simulink library "xbsIndex_r4"  (Simulink 7.1)
(part 3 of 9)

  "DDS v5_0 " : S-Function  LoadFcn=xlBlockLoadCallback(gcbh);  FunctionName=sysgen  Parameters=ptable_  EnableBusSupport=off  mask(Xilinx Direct Digital Synthesizer v5_0 Block){mode_sgadvanced=, mode=Sine, neg_sin_sgadvanced=, neg_sin=off, neg_cos_sgadvanced=, neg_cos=off, channels_sgadvanced=, channels=1, output_frequency_type_sgadvanced=, output_frequency_type=Fixed, output_frequency_array=[0.0], phase_offset_type_sgadvanced=, phase_offset_type=None, phase_offset_array=[0.0], channel_port_sgadvanced=, channel_port=off, rst_sgadvanced=, rst=off, en_sgadvanced=, en=on, explicit_period_sgadvanced=, explicit_period=on, period=1, dds_clock_rate=100.0, sfdr=36.0, frequency_resolution=0.4, acc_latency_sgadvanced=, acc_latency=One Cycle, noise_shaping_sgadvanced=, noise_shaping=None, dbl_ovrd_sgadvanced=, dbl_ovrd=off, mem_type_sgadvanced=, mem_type=Distributed Memory, pipeline_sgadvanced=, pipeline=off, use_rpm_sgadvanced=, use_rpm=on, xl_use_area_sgadvanced=, xl_use_area=off, xl_area=[0,0,0,0,0,0,0], has_advanced_control=0, sggui_pos=-1,-1,-1,-1, block_type=dds, block_version=, sg_icon_stat=60,60,-1,-1,white,blue,0,07734,right,,[ ],[ ], sg_mask_display=|, sg_list_contents=, sg_blockgui_xml=}
      mask sg_mask_display=|
      | fprintf('','COMMENT: begin icon graphics');
      | patch([0 60 60 0 0 ],[0 0 60 60 0 ],[0.77 0.82 0.91 ]);
      | plot([0 60 60 0 0 ],[0 0 60 60 0 ]);
      | patch([12.2 23.76 31.76 39.76 47.76 31.76 20.2 12.2 ],[38.88 38.88 46.88 38.88 46.88 46.88 46.88 38.88 ],[1 1 1 ]);
      | patch([20.2 31.76 23.76 12.2 20.2 ],[30.88 30.88 38.88 38.88 30.88 ],[0.931 0.946 0.973 ]);
      | patch([12.2 23.76 31.76 20.2 12.2 ],[22.88 22.88 30.88 30.88 22.88 ],[1 1 1 ]);
      | patch([20.2 47.76 39.76 31.76 23.76 12.2 20.2 ],[14.88 14.88 22.88 14.88 22.88 22.88 14.88 ],[0.931 0.946 0.973 ]);
      | fprintf('','COMMENT: end icon graphics');
      | fprintf('','COMMENT: begin icon text');
      | fprintf('','COMMENT: end icon text');
      mask prompts: mode_sgadvanced ""; mode "Function"; neg_sin_sgadvanced ""; neg_sin "Negative sine"; neg_cos_sgadvanced ""; neg_cos "Negative cosine"; channels_sgadvanced ""; output_frequency_type_sgadvanced ""; output_frequency_type "Type"; output_frequency_array "Output frequency array (MHz)"; phase_offset_type_sgadvanced ""; phase_offset_type "Type"; phase_offset_array "Phase offset angle array (x 2pi Radians)"; channel_port_sgadvanced ""; channel_port "Provide channel port"; rst_sgadvanced ""; rst "Provide synchronous reset port"; en_sgadvanced ""; en "Provide enable port"; explicit_period_sgadvanced ""; explicit_period "Sample period source"; period "Explicit period"; dds_clock_rate "DDS clock rate (MHz)"; sfdr "Spurious free dynamic range (dB)"; frequency_resolution "Frequency resolution (Hz)"; acc_latency_sgadvanced ""; acc_latency "Accumulator latency"; noise_shaping_sgadvanced ""; noise_shaping "Noise Shaping"; dbl_ovrd_sgadvanced ""; dbl_ovrd "Override with doubles"; mem_type_sgadvanced ""; mem_type "Memory type"; pipeline_sgadvanced ""; pipeline "Pipeline for maximum performance"; use_rpm_sgadvanced ""; use_rpm "Use core placement information"; xl_use_area_sgadvanced ""; xl_use_area "Define FPGA area for resource estimation"; xl_area "FPGA area [slices, FFs, BRAMs, LUTs, IOBs, emb. mults, TBUFs]"; has_advanced_control ""; sggui_pos ""; block_type ""; block_version ""; sg_icon_stat ""; sg_mask_display ""; sg_list_contents ""; sg_blockgui_xml ""
      mask help: Xilinx Direct Digital Synthesizer v5_0
      mask init:
      | try
      |   tmp_gcb = gcb;
      |   tmp_gcbh = gcbh;
      |   if (strcmp('SysGenIndex',get_param(bdroot(tmp_gcbh),'tag')) && ~isempty(regexp(bdroot(tmp_gcb), '^xbs', 'once')))
      |     return;
      |   end;
      |   xlMungeMaskParams;
      |   block_config = 'sysgen_blockset:Removed_config';
      | 
      |   block_type='dds';
      | nport = get_param(gcbh, 'ports');
      | nin = nport(1);
      | nout = nport(2);
      | 
      |   serialized_declarations = '{''acc_latency''=>''Int'',''channel_port''=>''Int'',''channels''=>''Int'',''dds_clock_rate''=>''Double'',''en''=>''Int'',''explicit_period''=>''Int'',''frequency_resolution''=>''Double'',''mem_type''=>''Int'',''mode''=>''Int'',''neg_cos''=>''Int'',''neg_sin''=>''Int'',''noise_shaping''=>''Int'',''output_frequency_array''=>''DoubleVector'',''output_frequency_type''=>''Int'',''period''=>''Double'',''phase_offset_array''=>''DoubleVector'',''phase_offset_type''=>''Int'',''pipeline''=>''Int'',''rst''=>''Int'',''sfdr''=>''Double'',''use_rpm''=>''Int'',''block_type''=>''String'',''nin''=>''Double'',''nout''=>''Double''}';
      |   ptable_ = xlblockprep(get_param(tmp_gcb, 'MaskWSVariables'));
      |   try
      |     xlBlockMoveCallback(tmp_gcbh);
      |   catch 
      |      clear global xl_updateicon_recursion_guard;
      |   end;
      | catch
      |   global dbgsysgen;
      |   if(~isempty(dbgsysgen) && dbgsysgen)
      |     e = regexprep(lasterr, '\n', '\nError: ');
      |     disp(['Error: While running MaskInit code on block ' tmp_gcb ': ' e]);
      |     error(e);
      |   end
      | end
      settings: CopyFcn=xlBlockMoveCallback(gcbh);  DeleteFcn=xlDestroyGui(gcbh);  ModelCloseFcn=xlDestroyGui(gcbh);  PreSaveFcn=xlBlockPreSaveCallback(gcbh);  PostSaveFcn=xlBlockPostSaveCallback(gcbh);  DestroyFcn=xlDestroyGui(gcbh);  OpenFcn=xlOpenGui(gcbh, 'dds_gui.xml', @xlremovedenablement, -1)  CloseFcn=xlDestroyGui(gcbh);  MoveFcn=xlBlockMoveCallback(gcbh);
      mask Help: eval('');xlDoc('-book','sysgen','-topic','DDS_v5_0');
      mask StyleString: edit,popup(Sine|Cosine|Sine and Cosine),edit,checkbox,edit,checkbox,edit,popup(1|2|3|4|5|6|7|8|9|10|11|12|13|14|15|16),edit,popup(Fixed|Programmable),edit,edit,popup(Fixed|Programmable|None),edit,edit,checkbox,edit,checkbox,edit,checkbox,edit,popup(on|off),edit,edit,edit,edit,edit,popup(Zero Cycle|One Cycle),edit,popup(None|Phase dithering|Taylor series corrected|Auto),edit,checkbox,edit,popup(Distributed Memory|Block RAM),edit,checkbox,edit,checkbox,edit,checkbox,edit,edit,edit,edit,edit,edit,edit,edit,edit
      mask Display:
      | fprintf('','COMMENT: begin icon graphics');
      | patch([0 60 60 0 0 ],[0 0 60 60 0 ],[0.77 0.82 0.91 ]);
      | plot([0 60 60 0 0 ],[0 0 60 60 0 ]);
      | patch([12.2 23.76 31.76 39.76 47.76 31.76 20.2 12.2 ],[38.88 38.88 46.88 38.88 46.88 46.88 46.88 38.88 ],[1 1 1 ]);
      | patch([20.2 31.76 23.76 12.2 20.2 ],[30.88 30.88 38.88 38.88 30.88 ],[0.931 0.946 0.973 ]);
      | patch([12.2 23.76 31.76 20.2 12.2 ],[22.88 22.88 30.88 30.88 22.88 ],[1 1 1 ]);
      | patch([20.2 47.76 39.76 31.76 23.76 12.2 20.2 ],[14.88 14.88 22.88 14.88 22.88 22.88 14.88 ],[0.931 0.946 0.973 ]);
      | fprintf('','COMMENT: end icon graphics');
      | fprintf('','COMMENT: begin icon text');
      | fprintf('','COMMENT: end icon text');
  DSP48 : S-Function  LoadFcn=xlBlockLoadCallback(gcbh);  FunctionName=sysgen  Parameters=ptable_  EnableBusSupport=off  mask(Xilinx DSP48 Block){use_b_sgadvanced=, use_b=Direct from B Port, use_op_sgadvanced=, use_op=off, use_creg_sgadvanced=, use_creg=off, use_pcin_sgadvanced=, use_pcin=off, use_pcout_sgadvanced=, use_pcout=off, use_bcout_sgadvanced=, use_bcout=off, rst_all_sgadvanced=, rst_all=off, en_all_sgadvanced=, en_all=off, pipeline_a_sgadvanced=, pipeline_a=1, pipeline_b_sgadvanced=, pipeline_b=1, pipeline_c_sgadvanced=, pipeline_c=on, pipeline_p_sgadvanced=, pipeline_p=on, pipeline_mult_sgadvanced=, pipeline_mult=on, pipeline_opmode_sgadvanced=, pipeline_opmode=on, pipeline_sub_sgadvanced=, pipeline_sub=on, pipeline_carryin_sgadvanced=, pipeline_carryin=on, pipeline_carryinsel_sgadvanced=, pipeline_carryinsel=on, rst_a_sgadvanced=, rst_a=off, rst_b_sgadvanced=, rst_b=off, rst_c_sgadvanced=, rst_c=off, rst_mult_sgadvanced=, rst_mult=off, rst_p_sgadvanced=, rst_p=off, rst_carry_in_sgadvanced=, rst_carry_in=off, rst_ctrl_sgadvanced=, rst_ctrl=off, en_a_sgadvanced=, en_a=off, en_b_sgadvanced=, en_b=off, en_c_sgadvanced=, en_c=off, en_mult_sgadvanced=, en_mult=off, en_p_sgadvanced=, en_p=off, en_carry_in_sgadvanced=, en_carry_in=off, en_ctrl_sgadvanced=, en_ctrl=off, dbl_ovrd_sgadvanced=, dbl_ovrd=off, use_synth_model_sgadvanced=, use_synth_model=off, xl_useadderonly_sgadvanced=, xl_useadderonly=off, xl_use_area_sgadvanced=, xl_use_area=off, xl_area=[0,0,0,0,0,0,0], has_advanced_control=0, sggui_pos=-1,-1,-1,-1, block_type=dsp48, block_version=, sg_icon_stat=75,136,6,1,white,blue,0,aaab5c39,right,,[ ],[ ], sg_mask_display=|, sg_list_contents=, sg_blockgui_xml=}
      mask sg_mask_display=|
      | fprintf('','COMMENT: begin icon graphics');
      | patch([0 75 75 0 0 ],[0 0 136 136 0 ],[0.77 0.82 0.91 ]);
      | plot([0 75 75 0 0 ],[0 0 136 136 0 ]);
      | patch([14.75 29.2 39.2 49.2 59.2 39.2 24.75 14.75 ],[79.1 79.1 89.1 79.1 89.1 89.1 89.1 79.1 ],[1 1 1 ]);
      | patch([24.75 39.2 29.2 14.75 24.75 ],[69.1 69.1 79.1 79.1 69.1 ],[0.931 0.946 0.973 ]);
      | patch([14.75 29.2 39.2 24.75 14.75 ],[59.1 59.1 69.1 69.1 59.1 ],[1 1 1 ]);
      | patch([24.75 59.2 49.2 39.2 29.2 14.75 24.75 ],[49.1 49.1 59.1 49.1 59.1 59.1 49.1 ],[0.931 0.946 0.973 ]);
      | fprintf('','COMMENT: end icon graphics');
      | fprintf('','COMMENT: begin icon text');
      | color('black');port_label('input',1,'a');
      | color('black');port_label('input',2,'b');
      | color('black');port_label('input',3,'opmode');
      | color('black');port_label('input',4,'subtract');
      | color('black');port_label('input',5,'carry_in');
      | color('black');port_label('input',6,'carry_in_sel');
      | color('black');port_label('output',1,'p');
      | fprintf('','COMMENT: end icon text');
      mask prompts: use_b_sgadvanced ""; use_b "<tt>B</tt> or <tt>BCIN</tt> input"; use_op_sgadvanced ""; use_op "Consolidate control port (<tt>opmode</tt>, <tt>subtract</tt>, <tt>carry_in</tt>, <tt>carry_in_sel</tt>)"; use_creg_sgadvanced ""; use_creg "Provide <tt>C</tt> port"; use_pcin_sgadvanced ""; use_pcin "Provide <tt>PCIN</tt> port"; use_pcout_sgadvanced ""; use_pcout "Provide <tt>PCOUT</tt> port"; use_bcout_sgadvanced ""; use_bcout "Provide <tt>BCOUT</tt> port"; rst_all_sgadvanced ""; rst_all "Provide global reset port"; en_all_sgadvanced ""; en_all "Provide global enable port"; pipeline_a_sgadvanced ""; pipeline_a "Length of <tt>A</tt> pipeline"; pipeline_b_sgadvanced ""; pipeline_b "Length of <tt>B</tt>/<tt>BCIN</tt> pipeline"; pipeline_c_sgadvanced ""; pipeline_c "Pipeline <tt>C</tt>"; pipeline_p_sgadvanced ""; pipeline_p "Pipeline <tt>P</tt>"; pipeline_mult_sgadvanced ""; pipeline_mult "Pipeline multiplier"; pipeline_opmode_sgadvanced ""; pipeline_opmode "Pipeline <tt>opmode</tt>"; pipeline_sub_sgadvanced ""; pipeline_sub "Pipeline <tt>subtract</tt>"; pipeline_carryin_sgadvanced ""; pipeline_carryin "Pipeline carry in"; pipeline_carryinsel_sgadvanced ""; pipeline_carryinsel "Pipeline carry in sel"; rst_a_sgadvanced ""; rst_a "Reset port for <tt>A</tt>"; rst_b_sgadvanced ""; rst_b "Reset port for <tt>B</tt>/<tt>BCIN</tt>"; rst_c_sgadvanced ""; rst_c "Reset port for <tt>C</tt>"; rst_mult_sgadvanced ""; rst_mult "Reset port for multiplier"; rst_p_sgadvanced ""; rst_p "Reset port for <tt>P</tt>"; rst_carry_in_sgadvanced ""; rst_carry_in "Reset port for carry in"; rst_ctrl_sgadvanced ""; rst_ctrl "Reset port for controls<br> (<tt>opmode</tt>, <tt>subtract</tt>,<br> <tt>carry_in</tt>, <tt>carry_in_sel</tt>)"; en_a_sgadvanced ""; en_a "Enable port for <tt>A</tt>"; en_b_sgadvanced ""; en_b "Enable port for <tt>B</tt>/<tt>BCIN</tt>"; en_c_sgadvanced ""; en_c "Enable port for <tt>C</tt>"; en_mult_sgadvanced ""; en_mult "Enable port for multiplier"; en_p_sgadvanced ""; en_p "Enable port for <tt>P</tt>"; en_carry_in_sgadvanced ""; en_carry_in "Enable port for carry in"; en_ctrl_sgadvanced ""; en_ctrl "Enable port for controls<br> (<tt>opmode</tt>, <tt>subtract</tt>,<br> <tt>carry_in</tt>, <tt>carry_in_sel</tt>)"; dbl_ovrd_sgadvanced ""; dbl_ovrd "Override with doubles"; use_synth_model_sgadvanced ""; use_synth_model "Use synthesizable model"; xl_useadderonly_sgadvanced ""; xl_useadderonly "Use adder only"; xl_use_area_sgadvanced ""; xl_use_area "Define FPGA area for resource estimation"; xl_area "FPGA area [slices, FFs, BRAMs, LUTs, IOBs, emb. mults, TBUFs]"; has_advanced_control ""; sggui_pos ""; block_type ""; block_version ""; sg_icon_stat ""; sg_mask_display ""; sg_list_contents ""; sg_blockgui_xml ""
      mask help: Xilinx DSP48
      mask init:
      | try
      |   tmp_gcb = gcb;
      |   tmp_gcbh = gcbh;
      |   if (strcmp('SysGenIndex',get_param(bdroot(tmp_gcbh),'tag')) && ~isempty(regexp(bdroot(tmp_gcb), '^xbs', 'once')))
      |     return;
      |   end;
      |   xlMungeMaskParams;
      |   block_config = 'sysgen_blockset:DSP48_config';
      | 
      |   block_type='dsp48';
      | 
      |   serialized_declarations = '{''en_a''=>''Int'',''en_all''=>''Int'',''en_b''=>''Int'',''en_c''=>''Int'',''en_carry_in''=>''Int'',''en_ctrl''=>''Int'',''en_mult''=>''Int'',''en_p''=>''Int'',''pipeline_a''=>''Int'',''pipeline_b''=>''Int'',''pipeline_c''=>''Int'',''pipeline_carryin''=>''Int'',''pipeline_carryinsel''=>''Int'',''pipeline_mult''=>''Int'',''pipeline_opmode''=>''Int'',''pipeline_p''=>''Int'',''pipeline_sub''=>''Int'',''rst_a''=>''Int'',''rst_all''=>''Int'',''rst_b''=>''Int'',''rst_c''=>''Int'',''rst_carry_in''=>''Int'',''rst_ctrl''=>''Int'',''rst_mult''=>''Int'',''rst_p''=>''Int'',''use_b''=>''Int'',''use_bcout''=>''Int'',''use_creg''=>''Int'',''use_op''=>''Int'',''use_pcin''=>''Int'',''use_pcout''=>''Int'',''use_synth_model''=>''Int'',''xl_useadderonly''=>''Int'',''block_type''=>''String''}';
      |   ptable_ = xlblockprep(get_param(tmp_gcb, 'MaskWSVariables'));
      |   try
      |     xlBlockMoveCallback(tmp_gcbh);
      |   catch 
      |      clear global xl_updateicon_recursion_guard;
      |   end;
      | catch
      |   global dbgsysgen;
      |   if(~isempty(dbgsysgen) && dbgsysgen)
      |     e = regexprep(lasterr, '\n', '\nError: ');
      |     disp(['Error: While running MaskInit code on block ' tmp_gcb ': ' e]);
      |     error(e);
      |   end
      | end
      settings: CopyFcn=xlBlockMoveCallback(gcbh);  DeleteFcn=xlDestroyGui(gcbh);  ModelCloseFcn=xlDestroyGui(gcbh);  PreSaveFcn=xlBlockPreSaveCallback(gcbh);  PostSaveFcn=xlBlockPostSaveCallback(gcbh);  DestroyFcn=xlDestroyGui(gcbh);  OpenFcn=xlOpenGui(gcbh, 'dsp48_gui.xml', @dsp48enablement, -1)  CloseFcn=xlDestroyGui(gcbh);  MoveFcn=xlBlockMoveCallback(gcbh);
      mask Help: eval('');xlDoc('-book','sysgen','-topic','DSP48');
      mask StyleString: edit,popup(Direct from B Port|Cascaded from BCIN Port),edit,checkbox,edit,checkbox,edit,checkbox,edit,checkbox,edit,checkbox,edit,checkbox,edit,checkbox,edit,popup(0|1|2),edit,popup(0|1|2),edit,checkbox,edit,checkbox,edit,checkbox,edit,checkbox,edit,checkbox,edit,checkbox,edit,checkbox,edit,checkbox,edit,checkbox,edit,checkbox,edit,checkbox,edit,checkbox,edit,checkbox,edit,checkbox,edit,checkbox,edit,checkbox,edit,checkbox,edit,checkbox,edit,checkbox,edit,checkbox,edit,checkbox,edit,checkbox,edit,checkbox,edit,checkbox,edit,checkbox,edit,edit,edit,edit,edit,edit,edit,edit,edit
      mask Display:
      | fprintf('','COMMENT: begin icon graphics');
      | patch([0 75 75 0 0 ],[0 0 136 136 0 ],[0.77 0.82 0.91 ]);
      | plot([0 75 75 0 0 ],[0 0 136 136 0 ]);
      | patch([14.75 29.2 39.2 49.2 59.2 39.2 24.75 14.75 ],[79.1 79.1 89.1 79.1 89.1 89.1 89.1 79.1 ],[1 1 1 ]);
      | patch([24.75 39.2 29.2 14.75 24.75 ],[69.1 69.1 79.1 79.1 69.1 ],[0.931 0.946 0.973 ]);
      | patch([14.75 29.2 39.2 24.75 14.75 ],[59.1 59.1 69.1 69.1 59.1 ],[1 1 1 ]);
      | patch([24.75 59.2 49.2 39.2 29.2 14.75 24.75 ],[49.1 49.1 59.1 49.1 59.1 59.1 49.1 ],[0.931 0.946 0.973 ]);
      | fprintf('','COMMENT: end icon graphics');
      | fprintf('','COMMENT: begin icon text');
      | color('black');port_label('input',1,'a');
      | color('black');port_label('input',2,'b');
      | color('black');port_label('input',3,'opmode');
      | color('black');port_label('input',4,'subtract');
      | color('black');port_label('input',5,'carry_in');
      | color('black');port_label('input',6,'carry_in_sel');
      | color('black');port_label('output',1,'p');
      | fprintf('','COMMENT: end icon text');
  DSP48 Macro : Subsystem  LoadFcn=xlBlockLoadCallback(gcbh);  mask(Xilinx DSP48 Macro Block){infoedit=Macro function to simplify use of the DSP48 primitive, especially as a dynamic operator, portalist=Xo, portblist=Yo, portclist=No, instrlist=|, pipeline_sgadvanced=, pipeline=Custom, pipeachoices_sgadvanced=, pipeachoices=1, pipebchoices_sgadvanced=, pipebchoices=1, pipecchoices_sgadvanced=, pipecchoices=on, pipepchoices_sgadvanced=, pipepchoices=on, pipemchoices_sgadvanced=, pipemchoices=on, pipectrlchoices_sgadvanced=, pipectrlchoices=on, pipemuxachoices_sgadvanced=, pipemuxachoices=0, pipemuxbchoices_sgadvanced=, pipemuxbchoices=0, pipemuxcchoices_sgadvanced=, pipemuxcchoices=0, pipemuxctrlchoices_sgadvanced=, pipemuxctrlchoices=0, pipeline_array_flag_sgadvanced=, pipeline_array_flag=off, custom_pipeline_cache=[1  1  1  1  1  1  0  0  0  0], precision_sgadvanced=, precision=Full, arith_type_sgadvanced=, arith_type=Unsigned, n_bits=8, bin_pt=2, bcout_sgadvanced=, bcout=off, acout_sgadvanced=, acout=off, carryout_sgadvanced=, carryout=off, carrycascout_sgadvanced=, carrycascout=off, pcout_sgadvanced=, pcout=off, rst_all_sgadvanced=, rst_all=off, rst_a_sgadvanced=, rst_a=off, rst_b_sgadvanced=, rst_b=off, rst_c_sgadvanced=, rst_c=off, rst_m_sgadvanced=, rst_m=off, rst_p_sgadvanced=, rst_p=off, rst_ctrl_sgadvanced=, rst_ctrl=off, ce_all_sgadvanced=, ce_all=off, ce_a_sgadvanced=, ce_a=off, ce_b_sgadvanced=, ce_b=off, ce_c_sgadvanced=, ce_c=off, ce_m_sgadvanced=, ce_m=off, ce_p_sgadvanced=, ce_p=off, ce_ctrl_sgadvanced=, ce_ctrl=off, dbl_ovrd_sgadvanced=, dbl_ovrd=off, synth_opt_sgadvanced=, synth_opt=on, errorlist=false, statestr=2d82c218ef9225b6e0048b8063710b3c, explicit_period=, period=1, maskdoc=, has_advanced_control=0, sggui_pos=-1,-1,-1,-1, block_type=dsp48macro, block_version=8.2.1, sg_icon_stat=90,138,3,1,white,blue,0,024d3c91cd129fc3834d91e223da5447,right,,[ ],[ ], sg_mask_display=|, sg_list_contents=, sg_blockgui_xml=}
      mask instrlist=|
      | <html><head><meta name="qrichtext" content="1" /></head><body style="font-size:8pt;font-family:MS Shell Dlg">
      | <p>P=Xo*Yo+No</p>
      | </body></html>
      mask sg_mask_display=|
      | fprintf('','COMMENT: begin icon graphics');
      | patch([0 90 90 0 0 ],[0 0 138 138 0 ],[0.77 0.82 0.91 ]);
      | plot([0 90 90 0 0 ],[0 0 138 138 0 ]);
      | patch([18.3 35.64 47.64 59.64 71.64 47.64 30.3 18.3 ],[82.32 82.32 94.32 82.32 94.32 94.32 94.32 82.32 ],[1 1 1 ]);
      | patch([30.3 47.64 35.64 18.3 30.3 ],[70.32 70.32 82.32 82.32 70.32 ],[0.931 0.946 0.973 ]);
      | patch([18.3 35.64 47.64 30.3 18.3 ],[58.32 58.32 70.32 70.32 58.32 ],[1 1 1 ]);
      | patch([30.3 71.64 59.64 47.64 35.64 18.3 30.3 ],[46.32 46.32 58.32 46.32 58.32 58.32 46.32 ],[0.931 0.946 0.973 ]);
      | fprintf('','COMMENT: end icon graphics');
      | fprintf('','COMMENT: begin icon text');
      | color('black');port_label('input',1,'Xo');
      | color('black');port_label('input',2,'Yo');
      | color('black');port_label('input',3,'No');
      | color('black');port_label('output',1,'P');
      | fprintf('','COMMENT: end icon text');
      mask prompts: infoedit ""; portalist "Inputs to port <tt>A</tt>"; portblist "Inputs to port <tt>B</tt>"; portclist "Inputs to port <tt>C</tt>"; instrlist "Instructions"; pipeline_sgadvanced ""; pipeline "Pipeline options"; pipeachoices_sgadvanced ""; pipeachoices "<tt>A</tt>"; pipebchoices_sgadvanced ""; pipebchoices "<tt>B</tt>"; pipecchoices_sgadvanced ""; pipecchoices "<tt>C</tt>"; pipepchoices_sgadvanced ""; pipepchoices "<tt>P</tt>"; pipemchoices_sgadvanced ""; pipemchoices "Multiplier"; pipectrlchoices_sgadvanced ""; pipectrlchoices "Controls (<tt>opmode</tt>, <tt>subtract</tt>,<br> <tt>carry_in</tt>, <tt>carry_in_sel</tt>)"; pipemuxachoices_sgadvanced ""; pipemuxachoices "MuxA"; pipemuxbchoices_sgadvanced ""; pipemuxbchoices "MuxB"; pipemuxcchoices_sgadvanced ""; pipemuxcchoices "MuxC"; pipemuxctrlchoices_sgadvanced ""; pipemuxctrlchoices "MuxCtrl"; pipeline_array_flag_sgadvanced ""; pipeline_array_flag "Define Using Array"; custom_pipeline_cache "Custom Pipeline Options([A,B,C,P,Ctrl,M,MuxA,MuxB,MuxC,MuxCtrl])"; precision_sgadvanced ""; arith_type_sgadvanced ""; arith_type "Output type"; n_bits "Number of bits"; bin_pt "Binary point"; bcout_sgadvanced ""; bcout "<tt>BCOUT</tt>"; acout_sgadvanced ""; acout "<tt>ACOUT</tt>"; carryout_sgadvanced ""; carryout "<tt>CARRYOUT</tt>"; carrycascout_sgadvanced ""; carrycascout "<tt>CARRYCASCOUT</tt>"; pcout_sgadvanced ""; pcout "<tt>PCOUT</tt>"; rst_all_sgadvanced ""; rst_all "<tt>Global Reset</tt>"; rst_a_sgadvanced ""; rst_a "Reset port for <tt>A</tt>"; rst_b_sgadvanced ""; rst_b "Reset port for <tt>B</tt>"; rst_c_sgadvanced ""; rst_c "Reset port for <tt>C</tt>"; rst_m_sgadvanced ""; rst_m "Reset port for multiplier"; rst_p_sgadvanced ""; rst_p "Reset port for <tt>P</tt>"; rst_ctrl_sgadvanced ""; rst_ctrl "Reset port for controls <br> (<tt>opmode</tt>, <tt>subtract</tt>,<br> <tt>carry_in</tt>, <tt>carry_in_sel</tt>)"; ce_all_sgadvanced ""; ce_all "<tt>Global Enable</tt>"; ce_a_sgadvanced ""; ce_a "Enable port for <tt>A</tt>"; ce_b_sgadvanced ""; ce_b "Enable port for <tt>B</tt>"; ce_c_sgadvanced ""; ce_c "Enable port for <tt>C</tt>"; ce_m_sgadvanced ""; ce_m "Enable port for multiplier"; ce_p_sgadvanced ""; ce_p "Enable port for <tt>P</tt>"; ce_ctrl_sgadvanced ""; ce_ctrl "Enable port for controls <br> (<tt>opmode</tt>, <tt>subtract</tt>,<br> <tt>carry_in</tt>, <tt>carry_in_sel</tt>)"; dbl_ovrd_sgadvanced ""; dbl_ovrd "Override with doubles"; synth_opt_sgadvanced ""; synth_opt "Use DSP48"; errorlist ""; statestr ""; explicit_period ""; period ""; maskdoc ""; has_advanced_control ""; sggui_pos ""; block_type ""; block_version ""; sg_icon_stat ""; sg_mask_display ""; sg_list_contents ""; sg_blockgui_xml ""
      mask help: Macro function to simplify use of the DSP48 primitive, especially as a dynamic operator
      mask init:
      | try
      |   tmp_gcb = gcb;
      |   tmp_gcbh = gcbh;
      |   if (strcmp('SysGenIndex',get_param(bdroot(tmp_gcbh),'tag')) && ~isempty(regexp(bdroot(tmp_gcb), '^xbs', 'once')))
      |     return;
      |   end;
      |   xlMungeMaskParams;
      | 
      |   block_type='dsp48macro';
      | 
      |   serialized_declarations = '{''block_type''=>''String''}';
      |   xldsp48macro_init();
      |   ptable_ = xlblockprep(get_param(tmp_gcb, 'MaskWSVariables'));
      |   try
      |     xlBlockMoveCallback(tmp_gcbh);
      |   catch 
      |      clear global xl_updateicon_recursion_guard;
      |   end;
      | catch
      |   global dbgsysgen;
      |   if(~isempty(dbgsysgen) && dbgsysgen)
      |     e = regexprep(lasterr, '\n', '\nError: ');
      |     disp(['Error: While running MaskInit code on block ' tmp_gcb ': ' e]);
      |     error(e);
      |   end
      | end
      settings: CopyFcn=tmp_gcbh = gcbh;set_param(tmp_gcbh,'linkstatus','none');xlBlockMoveCallback(gcbh);  DeleteFcn=xlDestroyGui(gcbh);  ModelCloseFcn=xlDestroyGui(gcbh);  PreSaveFcn=xlBlockPreSaveCallback(gcbh);  PostSaveFcn=xlBlockPostSaveCallback(gcbh);  DestroyFcn=xlDestroyGui(gcbh);  OpenFcn=xlOpenGui(gcbh, 'dsp48macro_gui.xml', @dsp48macroenablement, @dsp48macroaction)  CloseFcn=xlDestroyGui(gcbh);  MoveFcn=xlBlockMoveCallback(gcbh);
      mask Help: eval('');xlDoc('-book','sysgen','-topic','DSP48_Macro');
      mask StyleString: edit,edit,edit,edit,edit,edit,popup(External Registers|No External Registers|Custom),edit,popup(0|1|2),edit,popup(0|1|2),edit,checkbox,edit,checkbox,edit,checkbox,edit,checkbox,edit,popup(0|1|2),edit,popup(0|1|2),edit,popup(0|1|2),edit,popup(0|1|2),edit,checkbox,edit,edit,popup(Full|User Defined),edit,popup(Signed  (2's comp)|Unsigned),edit,edit,edit,checkbox,edit,checkbox,edit,checkbox,edit,checkbox,edit,checkbox,edit,checkbox,edit,checkbox,edit,checkbox,edit,checkbox,edit,checkbox,edit,checkbox,edit,checkbox,edit,checkbox,edit,checkbox,edit,checkbox,edit,checkbox,edit,checkbox,edit,checkbox,edit,checkbox,edit,checkbox,edit,checkbox,edit,edit,edit,edit,edit,edit,edit,edit,edit,edit,edit,edit,edit
      mask Display:
      | fprintf('','COMMENT: begin icon graphics');
      | patch([0 90 90 0 0 ],[0 0 138 138 0 ],[0.77 0.82 0.91 ]);
      | plot([0 90 90 0 0 ],[0 0 138 138 0 ]);
      | patch([18.3 35.64 47.64 59.64 71.64 47.64 30.3 18.3 ],[82.32 82.32 94.32 82.32 94.32 94.32 94.32 82.32 ],[1 1 1 ]);
      | patch([30.3 47.64 35.64 18.3 30.3 ],[70.32 70.32 82.32 82.32 70.32 ],[0.931 0.946 0.973 ]);
      | patch([18.3 35.64 47.64 30.3 18.3 ],[58.32 58.32 70.32 70.32 58.32 ],[1 1 1 ]);
      | patch([30.3 71.64 59.64 47.64 35.64 18.3 30.3 ],[46.32 46.32 58.32 46.32 58.32 58.32 46.32 ],[0.931 0.946 0.973 ]);
      | fprintf('','COMMENT: end icon graphics');
      | fprintf('','COMMENT: begin icon text');
      | color('black');port_label('input',1,'Xo');
      | color('black');port_label('input',2,'Yo');
      | color('black');port_label('input',3,'No');
      | color('black');port_label('output',1,'P');
      | fprintf('','COMMENT: end icon text');
  "DSP48 Macro 2.1 " : S-Function  LoadFcn=xlBlockLoadCallback(gcbh);  FunctionName=sysgen  Parameters=ptable_  EnableBusSupport=off  mask(Xilinx DSP48 Macro 2.1  Block){infoedit=<html>Valid operands: CONCAT, P, C, PCIN, P>>17, PCIN>>17, CARRYIN, CARRYCASCIN, ACIN, A, BCIN,B<br><br>Valid operators: +, -, *, ()<br><br>Valid functions: RNDSIMPLE, RNDSYM<br><br>Instructions are case insensitive and tolerate spaces.</html>, dsptype=, instruction_list=A*B+C, AvailableInstructions=A*B+C, show_filtered=off, pipeline_options=Automatic, dspimage=<html><img src="xbip_dsp48_macro_v2_1_regimag.png"></html>, tier_1=off, tier_2=off, tier_3=off, tier_4=off, tier_5=off, tier_6=off, dreg_1=off, dreg_2=off, dreg_3=off, areg_1=off, areg_2=off, areg_3=off, areg_4=off, breg_1=off, breg_2=off, breg_3=off, breg_4=off, mreg_5=off, concatreg_3=off, concatreg_4=off, concatreg_5=off, creg_1=off, creg_2=off, creg_3=off, creg_4=off, creg_5=off, preg_6=off, cinreg_1=off, cinreg_2=off, cinreg_3=off, cinreg_4=off, cinreg_5=off, opreg_1=off, opreg_2=off, opreg_3=off, opreg_4=off, opreg_5=off, output_properties=Full_Precision, p_width=48, p_binarywidth=0, has_acout=off, has_bcout=off, has_pcout=off, has_carryout=off, has_carrycascout=off, has_ce=off, has_d_ce=off, has_a_ce=off, has_b_ce=off, has_concat_ce=off, has_c_ce=off, has_m_ce=off, has_p_ce=off, has_sel_ce=off, has_sclr=off, has_d_sclr=off, has_a_sclr=off, has_b_sclr=off, has_concat_sclr=off, has_c_sclr=off, has_m_sclr=off, has_p_sclr=off, has_sel_sclr=off, use_dsp48_sgadvanced=, use_dsp48=on, gui_behaviour=Sysgen, instruction1=#, ip_name=DSP48 Macro, ip_version=2.1, dsptool_ready=true, ipcore_usecache=true, ipcore_useipmodelcache=true, wrapper_available=true, port_translation_map={ 'ce' => 'en', 'sclr' => 'rst'}, ipcore_xco_need_fpga_part=true, ipcore_fpga_part=xlipgetpartsetting(gcb, {'virtex6', 'xc6vlx75t', '-3', 'ff784'}), ipcore_latency_function='has_combinational', structural_sim=false, ipcore_verbose=false, ipcore_port_config={ 'carryin' => { 'arith' => 'ufix', 'binpt' => 0.00000000000, 'width' => 1.00000000000}, 'carrycascin' => { 'arith' => 'ufix', 'binpt' => 0.00000000000, 'width' => 1.00000000000}, 'carrycascout' => { 'arith' => 'ufix', 'binpt' => 0.00000000000, 'width' => 1.00000000000}, 'carryout' => { 'arith' => 'ufix', 'binpt' => 0.00000000000, 'width' => 1.00000000000}}, has_advanced_control=0, sggui_pos=-1,-1,-1,-1, block_type=xbip_dsp48_macro_v2_1, block_version=, sg_icon_stat=95,142,3,1,white,blue,0,c2be6e95,right,,[ ],[ ], sg_mask_display=|, sg_list_contents=, sg_blockgui_xml=}
      mask sg_mask_display=|
      | fprintf('','COMMENT: begin icon graphics');
      | patch([0 95 95 0 0 ],[0 0 142 142 0 ],[0.77 0.82 0.91 ]);
      | plot([0 95 95 0 0 ],[0 0 142 142 0 ]);
      | patch([18.075 36.86 49.86 62.86 75.86 49.86 31.075 18.075 ],[85.43 85.43 98.43 85.43 98.43 98.43 98.43 85.43 ],[1 1 1 ]);
      | patch([31.075 49.86 36.86 18.075 31.075 ],[72.43 72.43 85.43 85.43 72.43 ],[0.931 0.946 0.973 ]);
      | patch([18.075 36.86 49.86 31.075 18.075 ],[59.43 59.43 72.43 72.43 59.43 ],[1 1 1 ]);
      | patch([31.075 75.86 62.86 49.86 36.86 18.075 31.075 ],[46.43 46.43 59.43 46.43 59.43 59.43 46.43 ],[0.931 0.946 0.973 ]);
      | fprintf('','COMMENT: end icon graphics');
      | fprintf('','COMMENT: begin icon text');
      | color('black');port_label('input',1,'a');
      | color('black');port_label('input',2,'b');
      | color('black');port_label('input',3,'c');
      | color('black');port_label('output',1,'p');
      | fprintf('','COMMENT: end icon text');
      mask prompts: infoedit ""; dsptype ""; instruction_list ""; AvailableInstructions ""; show_filtered "Show Filtered Instructions"; pipeline_options "Pipeline Options"; dspimage ""; tier_1 "Tier 1"; tier_2 "Tier 2"; tier_3 "Tier 3"; tier_4 "Tier 4"; tier_5 "Tier 5"; tier_6 "Tier 6"; dreg_1 "D"; dreg_2 "D"; dreg_3 "D"; areg_1 "A"; areg_2 "A"; areg_3 "A"; areg_4 "A"; breg_1 "B"; breg_2 "B"; breg_3 "B"; breg_4 "B"; mreg_5 "M"; concatreg_3 "CONCAT"; concatreg_4 "CONCAT"; concatreg_5 "CONCAT"; creg_1 "C"; creg_2 "C"; creg_3 "C"; creg_4 "C"; creg_5 "C"; preg_6 "P"; cinreg_1 "CARRYIN"; cinreg_2 "CARRYIN"; cinreg_3 "CARRYIN"; cinreg_4 "CARRYIN"; cinreg_5 "CARRYIN"; opreg_1 "CONTROL"; opreg_2 "CONTROL"; opreg_3 "CONTROL"; opreg_4 "CONTROL"; opreg_5 "CONTROL"; output_properties ""; p_width "Width"; p_binarywidth "Binary Point"; has_acout "Use ACOUT"; has_bcout "Use BCOUT"; has_pcout "Use PCOUT"; has_carryout "Use CARRYOUT"; has_carrycascout "Use CARRYCASCOUT"; has_ce "Global"; has_d_ce "D"; has_a_ce "A"; has_b_ce "B"; has_concat_ce "CONCAT"; has_c_ce "C"; has_m_ce "M"; has_p_ce "P"; has_sel_ce "SEL/CARRYIN"; has_sclr "Global"; has_d_sclr "D"; has_a_sclr "A"; has_b_sclr "B"; has_concat_sclr "CONCAT"; has_c_sclr "C"; has_m_sclr "M"; has_p_sclr "P"; has_sel_sclr "SEL/CARRYIN"; use_dsp48_sgadvanced ""; use_dsp48 "Use XtremeDSP Slice"; gui_behaviour ""; instruction1 ""; ip_name ""; ip_version ""; dsptool_ready ""; ipcore_usecache ""; ipcore_useipmodelcache ""; wrapper_available ""; port_translation_map ""; ipcore_xco_need_fpga_part ""; ipcore_fpga_part ""; ipcore_latency_function ""; structural_sim ""; ipcore_verbose ""; ipcore_port_config ""; has_advanced_control ""; sggui_pos ""; block_type ""; block_version ""; sg_icon_stat ""; sg_mask_display ""; sg_list_contents ""; sg_blockgui_xml ""
      mask help:
      | Valid operands: CONCAT, P, C, PCIN, P>>17, PCIN>>17, CARRYIN, CARRYCASCIN, ACIN, A, BCIN,B
      |
      | Valid operators: +, -, *, ()
      |
      | Valid functions: RNDSIMPLE, RNDSYM
      |
      | Instructions are case insensitive and tolerate spaces.
      mask init:
      | try
      |   tmp_gcb = gcb;
      |   tmp_gcbh = gcbh;
      |   if (strcmp('SysGenIndex',get_param(bdroot(tmp_gcbh),'tag')) && ~isempty(regexp(bdroot(tmp_gcb), '^xbs', 'once')))
      |     return;
      |   end;
      |   xlMungeMaskParams;
      |   block_config = 'sysgen:coregenimport_config';
      | 
      |   block_type='xbip_dsp48_macro_v2_1';
      | 
      |   serialized_declarations = '{''AvailableInstructions''=>''String'',''areg_1''=>''Bool'',''areg_2''=>''Bool'',''areg_3''=>''Bool'',''areg_4''=>''Bool'',''breg_1''=>''Bool'',''breg_2''=>''Bool'',''breg_3''=>''Bool'',''breg_4''=>''Bool'',''cinreg_1''=>''Bool'',''cinreg_2''=>''Bool'',''cinreg_3''=>''Bool'',''cinreg_4''=>''Bool'',''cinreg_5''=>''Bool'',''concatreg_3''=>''Bool'',''concatreg_4''=>''Bool'',''concatreg_5''=>''Bool'',''creg_1''=>''Bool'',''creg_2''=>''Bool'',''creg_3''=>''Bool'',''creg_4''=>''Bool'',''creg_5''=>''Bool'',''dreg_1''=>''Bool'',''dreg_2''=>''Bool'',''dreg_3''=>''Bool'',''dsptool_ready''=>''Bool'',''gui_behaviour''=>''String'',''has_a_ce''=>''Bool'',''has_a_sclr''=>''Bool'',''has_acout''=>''Bool'',''has_b_ce''=>''Bool'',''has_b_sclr''=>''Bool'',''has_bcout''=>''Bool'',''has_c_ce''=>''Bool'',''has_c_sclr''=>''Bool'',''has_carrycascout''=>''Bool'',''has_carryout''=>''Bool'',''has_ce''=>''Bool'',''has_concat_ce''=>''Bool'',''has_concat_sclr''=>''Bool'',''has_d_ce''=>''Bool'',''has_d_sclr''=>''Bool'',''has_m_ce''=>''Bool'',''has_m_sclr''=>''Bool'',''has_p_ce''=>''Bool'',''has_p_sclr''=>''Bool'',''has_pcout''=>''Bool'',''has_sclr''=>''Bool'',''has_sel_ce''=>''Bool'',''has_sel_sclr''=>''Bool'',''instruction1''=>''String'',''instruction_list''=>''String'',''ip_name''=>''String'',''ip_version''=>''String'',''ipcore_fpga_part''=>''StringVector'',''ipcore_latency_function''=>''String'',''ipcore_port_config''=>''String'',''ipcore_usecache''=>''Bool'',''ipcore_useipmodelcache''=>''Bool'',''ipcore_verbose''=>''Bool'',''ipcore_xco_need_fpga_part''=>''Bool'',''mreg_5''=>''Bool'',''opreg_1''=>''Bool'',''opreg_2''=>''Bool'',''opreg_3''=>''Bool'',''opreg_4''=>''Bool'',''opreg_5''=>''Bool'',''output_properties''=>''String'',''p_binarywidth''=>''Int'',''p_width''=>''Int'',''pipeline_options''=>''String'',''port_translation_map''=>''String'',''preg_6''=>''Bool'',''show_filtered''=>''Bool'',''structural_sim''=>''Bool'',''tier_1''=>''Bool'',''tier_2''=>''Bool'',''tier_3''=>''Bool'',''tier_4''=>''Bool'',''tier_5''=>''Bool'',''tier_6''=>''Bool'',''use_dsp48''=>''Bool'',''wrapper_available''=>''Bool'',''block_type''=>''String''}';
      |   xlxbip_dsp48_macro_v2_1_init();
      |   ptable_ = xlblockprep(get_param(tmp_gcb, 'MaskWSVariables'));
      |   try
      |     xlBlockMoveCallback(tmp_gcbh);
      |   catch 
      |      clear global xl_updateicon_recursion_guard;
      |   end;
      | catch
      |   global dbgsysgen;
      |   if(~isempty(dbgsysgen) && dbgsysgen)
      |     e = regexprep(lasterr, '\n', '\nError: ');
      |     disp(['Error: While running MaskInit code on block ' tmp_gcb ': ' e]);
      |     error(e);
      |   end
      | end
      settings: CopyFcn=xlBlockMoveCallback(gcbh);  DeleteFcn=xlDestroyGui(gcbh);  ModelCloseFcn=xlDestroyGui(gcbh);  PreSaveFcn=xlBlockPreSaveCallback(gcbh);  PostSaveFcn=xlBlockPostSaveCallback(gcbh);  DestroyFcn=xlDestroyGui(gcbh);  OpenFcn=xlOpenGui(gcbh, 'xbip_dsp48_macro_v2_1_gui.xml', @xlxbip_dsp48_macro_v2_1_enablement, @xlxbip_dsp48_macro_v2_1_action)  CloseFcn=xlDestroyGui(gcbh);  MoveFcn=xlBlockMoveCallback(gcbh);
      mask Help: eval('');xlDoc('-book','sysgen','-topic','DSP48_Macro_2_1');
      mask StyleString: edit,edit,edit,edit,checkbox,popup(Automatic|By_Tier|Expert),edit,checkbox,checkbox,checkbox,checkbox,checkbox,checkbox,checkbox,checkbox,checkbox,checkbox,checkbox,checkbox,checkbox,checkbox,checkbox,checkbox,checkbox,checkbox,checkbox,checkbox,checkbox,checkbox,checkbox,checkbox,checkbox,checkbox,checkbox,checkbox,checkbox,checkbox,checkbox,checkbox,checkbox,checkbox,checkbox,checkbox,checkbox,popup(Full_Precision|User_Defined),edit,edit,checkbox,checkbox,checkbox,checkbox,checkbox,checkbox,checkbox,checkbox,checkbox,checkbox,checkbox,checkbox,checkbox,checkbox,checkbox,checkbox,checkbox,checkbox,checkbox,checkbox,checkbox,checkbox,checkbox,edit,checkbox,edit,edit,edit,edit,edit,edit,edit,edit,edit,edit,edit,edit,edit,edit,edit,edit,edit,edit,edit,edit,edit,edit,edit
      mask Display:
      | fprintf('','COMMENT: begin icon graphics');
      | patch([0 95 95 0 0 ],[0 0 142 142 0 ],[0.77 0.82 0.91 ]);
      | plot([0 95 95 0 0 ],[0 0 142 142 0 ]);
      | patch([18.075 36.86 49.86 62.86 75.86 49.86 31.075 18.075 ],[85.43 85.43 98.43 85.43 98.43 98.43 98.43 85.43 ],[1 1 1 ]);
      | patch([31.075 49.86 36.86 18.075 31.075 ],[72.43 72.43 85.43 85.43 72.43 ],[0.931 0.946 0.973 ]);
      | patch([18.075 36.86 49.86 31.075 18.075 ],[59.43 59.43 72.43 72.43 59.43 ],[1 1 1 ]);
      | patch([31.075 75.86 62.86 49.86 36.86 18.075 31.075 ],[46.43 46.43 59.43 46.43 59.43 59.43 46.43 ],[0.931 0.946 0.973 ]);
      | fprintf('','COMMENT: end icon graphics');
      | fprintf('','COMMENT: begin icon text');
      | color('black');port_label('input',1,'a');
      | color('black');port_label('input',2,'b');
      | color('black');port_label('input',3,'c');
      | color('black');port_label('output',1,'p');
      | fprintf('','COMMENT: end icon text');
  "DSP48 macro 2.0 " : S-Function  LoadFcn=xlBlockLoadCallback(gcbh);  FunctionName=sysgen  Parameters=ptable_  EnableBusSupport=off  mask(Xilinx DSP48 macro 2.0  Block){infoedit=<html>Valid operands: CONCAT, P, C, PCIN, P>>17, PCIN>>17, CARRYIN, CARRYCASCIN, ACIN, A, BCIN,B<br><br>Valid operators: +, -, *, ()<br><br>Valid functions: RNDSIMPLE, RNDSYM<br><br>Instructions are case insensitive and tolerate spaces.</html>, instruction_list=A*B+C, AvailableInstructions=A*B+C, show_filtered=off, pipeline_options=Automatic, dspimage=<html><img src="xbip_dsp48_macro_v2_0_regimag.png"></html>, tier_1=off, tier_2=off, tier_3=off, tier_4=off, tier_5=off, tier_6=off, dreg_1=off, dreg_2=off, dreg_3=off, areg_1=off, areg_2=off, areg_3=off, areg_4=off, breg_1=off, breg_2=off, breg_3=off, breg_4=off, mreg_5=off, concatreg_3=off, concatreg_4=off, concatreg_5=off, creg_1=off, creg_2=off, creg_3=off, creg_4=off, creg_5=off, preg_6=off, cinreg_1=off, cinreg_2=off, cinreg_3=off, cinreg_4=off, cinreg_5=off, opreg_1=off, opreg_2=off, opreg_3=off, opreg_4=off, opreg_5=off, output_properties=Full_Precision, p_width=48, p_binarywidth=0, has_carryout_sgadvanced=, has_carryout=off, has_acout_sgadvanced=, has_acout=off, has_bcout_sgadvanced=, has_bcout=off, has_carrycascout_sgadvanced=, has_carrycascout=off, has_pcout_sgadvanced=, has_pcout=off, has_ce_sgadvanced=, has_ce=off, has_sclr_sgadvanced=, has_sclr=off, use_dsp48_sgadvanced=, use_dsp48=on, gui_behaviour=Sysgen, instruction1=#, ip_name=DSP48 macro, ip_version=2.0, dsptool_ready=true, ipcore_usecache=true, ipcore_useipmodelcache=true, wrapper_available=true, port_translation_map={ 'ce' => 'en', 'sclr' => 'rst'}, ipcore_xco_need_fpga_part=true, ipcore_fpga_part=xlipgetpartsetting(gcb, {'virtex4', 'xc4vsx35', '-10', 'ff668'}), ipcore_latency_function='has_combinational', structural_sim=false, ipcore_verbose=false, ipcore_port_config={ 'carryin' => { 'arith' => 'ufix', 'binpt' => 0.00000000000, 'width' => 1.00000000000}, 'carrycascin' => { 'arith' => 'ufix', 'binpt' => 0.00000000000, 'width' => 1.00000000000}, 'carrycascout' => { 'arith' => 'ufix', 'binpt' => 0.00000000000, 'width' => 1.00000000000}, 'carryout' => { 'arith' => 'ufix', 'binpt' => 0.00000000000, 'width' => 1.00000000000}}, has_advanced_control=0, sggui_pos=-1,-1,-1,-1, block_type=xbip_dsp48_macro_v2_0, block_version=, sg_icon_stat=95,142,3,1,white,blue,0,c2be6e95,right,,[ ],[ ], sg_mask_display=|, sg_list_contents=, sg_blockgui_xml=}
      mask sg_mask_display=|
      | fprintf('','COMMENT: begin icon graphics');
      | patch([0 95 95 0 0 ],[0 0 142 142 0 ],[0.77 0.82 0.91 ]);
      | plot([0 95 95 0 0 ],[0 0 142 142 0 ]);
      | patch([18.075 36.86 49.86 62.86 75.86 49.86 31.075 18.075 ],[85.43 85.43 98.43 85.43 98.43 98.43 98.43 85.43 ],[1 1 1 ]);
      | patch([31.075 49.86 36.86 18.075 31.075 ],[72.43 72.43 85.43 85.43 72.43 ],[0.931 0.946 0.973 ]);
      | patch([18.075 36.86 49.86 31.075 18.075 ],[59.43 59.43 72.43 72.43 59.43 ],[1 1 1 ]);
      | patch([31.075 75.86 62.86 49.86 36.86 18.075 31.075 ],[46.43 46.43 59.43 46.43 59.43 59.43 46.43 ],[0.931 0.946 0.973 ]);
      | fprintf('','COMMENT: end icon graphics');
      | fprintf('','COMMENT: begin icon text');
      | color('black');port_label('input',1,'a');
      | color('black');port_label('input',2,'b');
      | color('black');port_label('input',3,'c');
      | color('black');port_label('output',1,'p');
      | fprintf('','COMMENT: end icon text');
      mask prompts: infoedit ""; instruction_list ""; AvailableInstructions ""; show_filtered "Show Filtered Instructions"; pipeline_options "Pipeline Options"; dspimage ""; tier_1 "Tier 1"; tier_2 "Tier 2"; tier_3 "Tier 3"; tier_4 "Tier 4"; tier_5 "Tier 5"; tier_6 "Tier 6"; dreg_1 "D"; dreg_2 "D"; dreg_3 "D"; areg_1 "A"; areg_2 "A"; areg_3 "A"; areg_4 "A"; breg_1 "B"; breg_2 "B"; breg_3 "B"; breg_4 "B"; mreg_5 "M"; concatreg_3 "CONCAT"; concatreg_4 "CONCAT"; concatreg_5 "CONCAT"; creg_1 "C"; creg_2 "C"; creg_3 "C"; creg_4 "C"; creg_5 "C"; preg_6 "P"; cinreg_1 "CARRYIN"; cinreg_2 "CARRYIN"; cinreg_3 "CARRYIN"; cinreg_4 "CARRYIN"; cinreg_5 "CARRYIN"; opreg_1 "CONTROL"; opreg_2 "CONTROL"; opreg_3 "CONTROL"; opreg_4 "CONTROL"; opreg_5 "CONTROL"; output_properties ""; p_width "Width"; p_binarywidth "Binary Point"; has_carryout_sgadvanced ""; has_carryout "Use CARRYOUT"; has_acout_sgadvanced ""; has_acout "Use ACOUT"; has_bcout_sgadvanced ""; has_bcout "Use BCOUT"; has_carrycascout_sgadvanced ""; has_carrycascout "Use CARRYCASCOUT"; has_pcout_sgadvanced ""; has_pcout "Use PCOUT"; has_ce_sgadvanced ""; has_ce "en"; has_sclr_sgadvanced ""; has_sclr "rst"; use_dsp48_sgadvanced ""; use_dsp48 "Use XtremeDSP Slice"; gui_behaviour ""; instruction1 ""; ip_name ""; ip_version ""; dsptool_ready ""; ipcore_usecache ""; ipcore_useipmodelcache ""; wrapper_available ""; port_translation_map ""; ipcore_xco_need_fpga_part ""; ipcore_fpga_part ""; ipcore_latency_function ""; structural_sim ""; ipcore_verbose ""; ipcore_port_config ""; has_advanced_control ""; sggui_pos ""; block_type ""; block_version ""; sg_icon_stat ""; sg_mask_display ""; sg_list_contents ""; sg_blockgui_xml ""
      mask help:
      | Valid operands: CONCAT, P, C, PCIN, P>>17, PCIN>>17, CARRYIN, CARRYCASCIN, ACIN, A, BCIN,B
      |
      | Valid operators: +, -, *, ()
      |
      | Valid functions: RNDSIMPLE, RNDSYM
      |
      | Instructions are case insensitive and tolerate spaces.
      mask init:
      | try
      |   tmp_gcb = gcb;
      |   tmp_gcbh = gcbh;
      |   if (strcmp('SysGenIndex',get_param(bdroot(tmp_gcbh),'tag')) && ~isempty(regexp(bdroot(tmp_gcb), '^xbs', 'once')))
      |     return;
      |   end;
      |   xlMungeMaskParams;
      |   block_config = 'sysgen:coregenimport_config';
      | 
      |   block_type='xbip_dsp48_macro_v2_0';
      | 
      |   serialized_declarations = '{''AvailableInstructions''=>''String'',''areg_1''=>''Bool'',''areg_2''=>''Bool'',''areg_3''=>''Bool'',''areg_4''=>''Bool'',''breg_1''=>''Bool'',''breg_2''=>''Bool'',''breg_3''=>''Bool'',''breg_4''=>''Bool'',''cinreg_1''=>''Bool'',''cinreg_2''=>''Bool'',''cinreg_3''=>''Bool'',''cinreg_4''=>''Bool'',''cinreg_5''=>''Bool'',''concatreg_3''=>''Bool'',''concatreg_4''=>''Bool'',''concatreg_5''=>''Bool'',''creg_1''=>''Bool'',''creg_2''=>''Bool'',''creg_3''=>''Bool'',''creg_4''=>''Bool'',''creg_5''=>''Bool'',''dreg_1''=>''Bool'',''dreg_2''=>''Bool'',''dreg_3''=>''Bool'',''dsptool_ready''=>''Bool'',''gui_behaviour''=>''String'',''has_acout''=>''Bool'',''has_bcout''=>''Bool'',''has_carrycascout''=>''Bool'',''has_carryout''=>''Bool'',''has_ce''=>''Bool'',''has_pcout''=>''Bool'',''has_sclr''=>''Bool'',''instruction1''=>''String'',''instruction_list''=>''String'',''ip_name''=>''String'',''ip_version''=>''String'',''ipcore_fpga_part''=>''StringVector'',''ipcore_latency_function''=>''String'',''ipcore_port_config''=>''String'',''ipcore_usecache''=>''Bool'',''ipcore_useipmodelcache''=>''Bool'',''ipcore_verbose''=>''Bool'',''ipcore_xco_need_fpga_part''=>''Bool'',''mreg_5''=>''Bool'',''opreg_1''=>''Bool'',''opreg_2''=>''Bool'',''opreg_3''=>''Bool'',''opreg_4''=>''Bool'',''opreg_5''=>''Bool'',''output_properties''=>''String'',''p_binarywidth''=>''Int'',''p_width''=>''Int'',''pipeline_options''=>''String'',''port_translation_map''=>''String'',''preg_6''=>''Bool'',''show_filtered''=>''Bool'',''structural_sim''=>''Bool'',''tier_1''=>''Bool'',''tier_2''=>''Bool'',''tier_3''=>''Bool'',''tier_4''=>''Bool'',''tier_5''=>''Bool'',''tier_6''=>''Bool'',''use_dsp48''=>''Bool'',''wrapper_available''=>''Bool'',''block_type''=>''String''}';
      |   xlxbip_dsp48_macro_v2_0_init();
      |   ptable_ = xlblockprep(get_param(tmp_gcb, 'MaskWSVariables'));
      |   try
      |     xlBlockMoveCallback(tmp_gcbh);
      |   catch 
      |      clear global xl_updateicon_recursion_guard;
      |   end;
      | catch
      |   global dbgsysgen;
      |   if(~isempty(dbgsysgen) && dbgsysgen)
      |     e = regexprep(lasterr, '\n', '\nError: ');
      |     disp(['Error: While running MaskInit code on block ' tmp_gcb ': ' e]);
      |     error(e);
      |   end
      | end
      settings: CopyFcn=xlBlockMoveCallback(gcbh);  DeleteFcn=xlDestroyGui(gcbh);  ModelCloseFcn=xlDestroyGui(gcbh);  PreSaveFcn=xlBlockPreSaveCallback(gcbh);  PostSaveFcn=xlBlockPostSaveCallback(gcbh);  DestroyFcn=xlDestroyGui(gcbh);  OpenFcn=xlOpenGui(gcbh, 'xbip_dsp48_macro_v2_0_gui.xml', @xlxbip_dsp48_macro_v2_0_enablement, @xlxbip_dsp48_macro_v2_0_action)  CloseFcn=xlDestroyGui(gcbh);  MoveFcn=xlBlockMoveCallback(gcbh);
      mask Help: eval('');xlDoc('-book','sysgen','-topic','DSP48_macro_2_0');
      mask StyleString: edit,edit,edit,checkbox,popup(Automatic|By_Tier|Expert),edit,checkbox,checkbox,checkbox,checkbox,checkbox,checkbox,checkbox,checkbox,checkbox,checkbox,checkbox,checkbox,checkbox,checkbox,checkbox,checkbox,checkbox,checkbox,checkbox,checkbox,checkbox,checkbox,checkbox,checkbox,checkbox,checkbox,checkbox,checkbox,checkbox,checkbox,checkbox,checkbox,checkbox,checkbox,checkbox,checkbox,checkbox,popup(Full_Precision|User_Defined),edit,edit,edit,checkbox,edit,checkbox,edit,checkbox,edit,checkbox,edit,checkbox,edit,checkbox,edit,checkbox,edit,checkbox,edit,edit,edit,edit,edit,edit,edit,edit,edit,edit,edit,edit,edit,edit,edit,edit,edit,edit,edit,edit,edit,edit,edit
      mask Display:
      | fprintf('','COMMENT: begin icon graphics');
      | patch([0 95 95 0 0 ],[0 0 142 142 0 ],[0.77 0.82 0.91 ]);
      | plot([0 95 95 0 0 ],[0 0 142 142 0 ]);
      | patch([18.075 36.86 49.86 62.86 75.86 49.86 31.075 18.075 ],[85.43 85.43 98.43 85.43 98.43 98.43 98.43 85.43 ],[1 1 1 ]);
      | patch([31.075 49.86 36.86 18.075 31.075 ],[72.43 72.43 85.43 85.43 72.43 ],[0.931 0.946 0.973 ]);
      | patch([18.075 36.86 49.86 31.075 18.075 ],[59.43 59.43 72.43 72.43 59.43 ],[1 1 1 ]);
      | patch([31.075 75.86 62.86 49.86 36.86 18.075 31.075 ],[46.43 46.43 59.43 46.43 59.43 59.43 46.43 ],[0.931 0.946 0.973 ]);
      | fprintf('','COMMENT: end icon graphics');
      | fprintf('','COMMENT: begin icon text');
      | color('black');port_label('input',1,'a');
      | color('black');port_label('input',2,'b');
      | color('black');port_label('input',3,'c');
      | color('black');port_label('output',1,'p');
      | fprintf('','COMMENT: end icon text');
  DSP48A : S-Function  LoadFcn=xlBlockLoadCallback(gcbh);  FunctionName=sysgen  Parameters=ptable_  EnableBusSupport=off  mask(Xilinx DSP48A Block){use_op_sgadvanced=, use_op=on, use_creg_sgadvanced=, use_creg=off, use_d_sgadvanced=, use_d=off, use_pcin_sgadvanced=, use_pcin=off, use_pcout_sgadvanced=, use_pcout=off, use_bcout_sgadvanced=, use_bcout=off, use_carryin_sgadvanced=, use_carryin=off, use_carryout_sgadvanced=, use_carryout=off, rst_all_sgadvanced=, rst_all=off, en_all_sgadvanced=, en_all=off, carryin_type_sgadvanced=, carryin_type=Direct from carry in port, use_a0reg_sgadvanced=, use_a0reg=on, use_a1reg_sgadvanced=, use_a1reg=on, use_b0reg_sgadvanced=, use_b0reg=on, use_b1reg_sgadvanced=, use_b1reg=on, pipeline_c_sgadvanced=, pipeline_c=on, pipeline_d_sgadvanced=, pipeline_d=on, pipeline_mult_sgadvanced=, pipeline_mult=on, pipeline_p_sgadvanced=, pipeline_p=on, pipeline_opmode_sgadvanced=, pipeline_opmode=on, pipeline_carryin_sgadvanced=, pipeline_carryin=on, rst_a_sgadvanced=, rst_a=off, rst_b_sgadvanced=, rst_b=off, rst_c_sgadvanced=, rst_c=off, rst_d_sgadvanced=, rst_d=off, rst_mult_sgadvanced=, rst_mult=off, rst_p_sgadvanced=, rst_p=off, rst_opmode_sgadvanced=, rst_opmode=off, rst_carry_in_sgadvanced=, rst_carry_in=off, en_a_sgadvanced=, en_a=off, en_b_sgadvanced=, en_b=off, en_c_sgadvanced=, en_c=off, en_d_sgadvanced=, en_d=off, en_mult_sgadvanced=, en_mult=off, en_p_sgadvanced=, en_p=off, en_opmode_sgadvanced=, en_opmode=off, en_carry_in_sgadvanced=, en_carry_in=off, dbl_ovrd_sgadvanced=, dbl_ovrd=off, use_synth_model_sgadvanced=, use_synth_model=off, xl_use_area_sgadvanced=, xl_use_area=off, xl_area=[0,0,0,0,0,0,0], device=3, has_advanced_control=0, sggui_pos=-1,-1,-1,-1, block_type=dsp48a, block_version=, sg_icon_stat=75,136,3,1,white,blue,0,b50c3739,right,,[ ],[ ], sg_mask_display=|, sg_list_contents=, sg_blockgui_xml=}
      mask sg_mask_display=|
      | fprintf('','COMMENT: begin icon graphics');
      | patch([0 75 75 0 0 ],[0 0 136 136 0 ],[0.77 0.82 0.91 ]);
      | plot([0 75 75 0 0 ],[0 0 136 136 0 ]);
      | patch([14.75 29.2 39.2 49.2 59.2 39.2 24.75 14.75 ],[79.1 79.1 89.1 79.1 89.1 89.1 89.1 79.1 ],[1 1 1 ]);
      | patch([24.75 39.2 29.2 14.75 24.75 ],[69.1 69.1 79.1 79.1 69.1 ],[0.931 0.946 0.973 ]);
      | patch([14.75 29.2 39.2 24.75 14.75 ],[59.1 59.1 69.1 69.1 59.1 ],[1 1 1 ]);
      | patch([24.75 59.2 49.2 39.2 29.2 14.75 24.75 ],[49.1 49.1 59.1 49.1 59.1 59.1 49.1 ],[0.931 0.946 0.973 ]);
      | fprintf('','COMMENT: end icon graphics');
      | fprintf('','COMMENT: begin icon text');
      | color('black');port_label('input',1,'a');
      | color('black');port_label('input',2,'b');
      | color('black');port_label('input',3,'op');
      | color('black');port_label('output',1,'p');
      | fprintf('','COMMENT: end icon text');
      mask prompts: use_op_sgadvanced ""; use_op "Consolidate control port (opmode, carry_in, preadd select, preadd subtract)"; use_creg_sgadvanced ""; use_creg "Provide <tt>C</tt> port"; use_d_sgadvanced ""; use_d "Provide <tt>D</tt> port"; use_pcin_sgadvanced ""; use_pcin "Provide <tt>PCIN</tt> port"; use_pcout_sgadvanced ""; use_pcout "Provide <tt>PCOUT</tt> port"; use_bcout_sgadvanced ""; use_bcout "Provide <tt>BCOUT</tt> port"; use_carryin_sgadvanced ""; use_carryin "Provide <tt>CARRYIN</tt> port"; use_carryout_sgadvanced ""; use_carryout "Provide <tt>CARRYOUT</tt> port"; rst_all_sgadvanced ""; rst_all "Provide global reset port"; en_all_sgadvanced ""; en_all "Provide global enable port"; carryin_type_sgadvanced ""; carryin_type "Carry in input"; use_a0reg_sgadvanced ""; use_a0reg "Use A0 reg"; use_a1reg_sgadvanced ""; use_a1reg "Use A1 reg"; use_b0reg_sgadvanced ""; use_b0reg "Use B0 reg"; use_b1reg_sgadvanced ""; use_b1reg "Use B1 reg"; pipeline_c_sgadvanced ""; pipeline_c "Pipeline <tt>C</tt>"; pipeline_d_sgadvanced ""; pipeline_d "Pipeline <tt>D</tt>"; pipeline_mult_sgadvanced ""; pipeline_mult "Pipeline multiplier"; pipeline_p_sgadvanced ""; pipeline_p "Pipeline <tt>P</tt>"; pipeline_opmode_sgadvanced ""; pipeline_opmode "Pipeline <tt>opmode</tt>"; pipeline_carryin_sgadvanced ""; pipeline_carryin "Pipeline carry in"; rst_a_sgadvanced ""; rst_a "Reset port for <tt>A</tt>"; rst_b_sgadvanced ""; rst_b "Reset port for <tt>B</tt>"; rst_c_sgadvanced ""; rst_c "Reset port for <tt>C</tt>"; rst_d_sgadvanced ""; rst_d "Reset port for <tt>D</tt>"; rst_mult_sgadvanced ""; rst_mult "Reset port for multiplier"; rst_p_sgadvanced ""; rst_p "Reset port for <tt>P</tt>"; rst_opmode_sgadvanced ""; rst_opmode "Reset port for <tt>opmode</tt>"; rst_carry_in_sgadvanced ""; rst_carry_in "Reset port for carry in"; en_a_sgadvanced ""; en_a "Enable port for <tt>A</tt>"; en_b_sgadvanced ""; en_b "Enable port for <tt>B</tt>"; en_c_sgadvanced ""; en_c "Enable port for <tt>C</tt>"; en_d_sgadvanced ""; en_d "Enable port for <tt>D</tt>"; en_mult_sgadvanced ""; en_mult "Enable port for multiplier"; en_p_sgadvanced ""; en_p "Enable port for <tt>P</tt>"; en_opmode_sgadvanced ""; en_opmode "Enable port for <tt>opmode</tt>"; en_carry_in_sgadvanced ""; en_carry_in "Enable port for carry in"; dbl_ovrd_sgadvanced ""; dbl_ovrd "Override with doubles"; use_synth_model_sgadvanced ""; use_synth_model "Use synthesizable model"; xl_use_area_sgadvanced ""; xl_use_area "Define FPGA area for resource estimation"; xl_area "FPGA area [slices, FFs, BRAMs, LUTs, IOBs, emb. mults, TBUFs]"; device ""; has_advanced_control ""; sggui_pos ""; block_type ""; block_version ""; sg_icon_stat ""; sg_mask_display ""; sg_list_contents ""; sg_blockgui_xml ""
      mask help: Xilinx DSP48A
      mask init:
      | try
      |   tmp_gcb = gcb;
      |   tmp_gcbh = gcbh;
      |   if (strcmp('SysGenIndex',get_param(bdroot(tmp_gcbh),'tag')) && ~isempty(regexp(bdroot(tmp_gcb), '^xbs', 'once')))
      |     return;
      |   end;
      |   xlMungeMaskParams;
      |   block_config = 'sysgen_blockset:DSP48A_config';
      | 
      |   block_type='dsp48a';
      | 
      |   serialized_declarations = '{''carryin_type''=>''Int'',''dbl_ovrd''=>''Bool'',''device''=>''Int'',''en_a''=>''Bool'',''en_all''=>''Bool'',''en_b''=>''Bool'',''en_c''=>''Bool'',''en_carry_in''=>''Bool'',''en_d''=>''Bool'',''en_mult''=>''Bool'',''en_opmode''=>''Bool'',''en_p''=>''Bool'',''pipeline_c''=>''Bool'',''pipeline_carryin''=>''Bool'',''pipeline_d''=>''Bool'',''pipeline_mult''=>''Bool'',''pipeline_opmode''=>''Bool'',''pipeline_p''=>''Bool'',''rst_a''=>''Bool'',''rst_all''=>''Bool'',''rst_b''=>''Bool'',''rst_c''=>''Bool'',''rst_carry_in''=>''Bool'',''rst_d''=>''Bool'',''rst_mult''=>''Bool'',''rst_opmode''=>''Bool'',''rst_p''=>''Bool'',''use_a0reg''=>''Bool'',''use_a1reg''=>''Bool'',''use_b0reg''=>''Bool'',''use_b1reg''=>''Bool'',''use_bcout''=>''Bool'',''use_carryin''=>''Bool'',''use_carryout''=>''Bool'',''use_creg''=>''Bool'',''use_d''=>''Bool'',''use_op''=>''Bool'',''use_pcin''=>''Bool'',''use_pcout''=>''Bool'',''use_synth_model''=>''Bool'',''block_type''=>''String''}';
      |   ptable_ = xlblockprep(get_param(tmp_gcb, 'MaskWSVariables'));
      |   try
      |     xlBlockMoveCallback(tmp_gcbh);
      |   catch 
      |      clear global xl_updateicon_recursion_guard;
      |   end;
      | catch
      |   global dbgsysgen;
      |   if(~isempty(dbgsysgen) && dbgsysgen)
      |     e = regexprep(lasterr, '\n', '\nError: ');
      |     disp(['Error: While running MaskInit code on block ' tmp_gcb ': ' e]);
      |     error(e);
      |   end
      | end
      settings: CopyFcn=xlBlockMoveCallback(gcbh);  DeleteFcn=xlDestroyGui(gcbh);  ModelCloseFcn=xlDestroyGui(gcbh);  PreSaveFcn=xlBlockPreSaveCallback(gcbh);  PostSaveFcn=xlBlockPostSaveCallback(gcbh);  DestroyFcn=xlDestroyGui(gcbh);  OpenFcn=xlOpenGui(gcbh, 'dsp48a_gui.xml', @dsp48aenablement, -1)  CloseFcn=xlDestroyGui(gcbh);  MoveFcn=xlBlockMoveCallback(gcbh);
      mask Help: eval('');xlDoc('-book','sysgen','-topic','DSP48A');
      mask StyleString: edit,checkbox,edit,checkbox,edit,checkbox,edit,checkbox,edit,checkbox,edit,checkbox,edit,checkbox,edit,checkbox,edit,checkbox,edit,checkbox,edit,popup(Direct from carry in port|Cascaded from carry in port),edit,checkbox,edit,checkbox,edit,checkbox,edit,checkbox,edit,checkbox,edit,checkbox,edit,checkbox,edit,checkbox,edit,checkbox,edit,checkbox,edit,checkbox,edit,checkbox,edit,checkbox,edit,checkbox,edit,checkbox,edit,checkbox,edit,checkbox,edit,checkbox,edit,checkbox,edit,checkbox,edit,checkbox,edit,checkbox,edit,checkbox,edit,checkbox,edit,checkbox,edit,checkbox,edit,checkbox,edit,checkbox,edit,checkbox,edit,edit,edit,edit,edit,edit,edit,edit,edit,edit
      mask Display:
      | fprintf('','COMMENT: begin icon graphics');
      | patch([0 75 75 0 0 ],[0 0 136 136 0 ],[0.77 0.82 0.91 ]);
      | plot([0 75 75 0 0 ],[0 0 136 136 0 ]);
      | patch([14.75 29.2 39.2 49.2 59.2 39.2 24.75 14.75 ],[79.1 79.1 89.1 79.1 89.1 89.1 89.1 79.1 ],[1 1 1 ]);
      | patch([24.75 39.2 29.2 14.75 24.75 ],[69.1 69.1 79.1 79.1 69.1 ],[0.931 0.946 0.973 ]);
      | patch([14.75 29.2 39.2 24.75 14.75 ],[59.1 59.1 69.1 69.1 59.1 ],[1 1 1 ]);
      | patch([24.75 59.2 49.2 39.2 29.2 14.75 24.75 ],[49.1 49.1 59.1 49.1 59.1 59.1 49.1 ],[0.931 0.946 0.973 ]);
      | fprintf('','COMMENT: end icon graphics');
      | fprintf('','COMMENT: begin icon text');
      | color('black');port_label('input',1,'a');
      | color('black');port_label('input',2,'b');
      | color('black');port_label('input',3,'op');
      | color('black');port_label('output',1,'p');
      | fprintf('','COMMENT: end icon text');
  DSP48E : S-Function  LoadFcn=xlBlockLoadCallback(gcbh);  FunctionName=sysgen  Parameters=ptable_  EnableBusSupport=off  mask(Xilinx DSP48E Block){use_a_sgadvanced=, use_a=Direct from A Port, use_b_sgadvanced=, use_b=Direct from B Port, reset_preg_sgadvanced=, reset_preg=off, pattern_from_creg_sgadvanced=, pattern_from_creg=on, pattern='000000000000', mask_from_creg_sgadvanced=, mask_from_creg=on, pattern_mask='000000000000', sel_rounding_mask_sgadvanced=, sel_rounding_mask=Select mask, use_op_sgadvanced=, use_op=off, use_creg_sgadvanced=, use_creg=off, rst_all_sgadvanced=, rst_all=off, en_all_sgadvanced=, en_all=off, use_pcin_sgadvanced=, use_pcin=off, use_carrycascin_sgadvanced=, use_carrycascin=off, use_multsignin_sgadvanced=, use_multsignin=off, use_carryout_sgadvanced=, use_carryout=off, use_patterndetect_sgadvanced=, use_patterndetect=off, use_patternbdetect_sgadvanced=, use_patternbdetect=off, use_overflow_sgadvanced=, use_overflow=off, use_underflow_sgadvanced=, use_underflow=off, use_acout_sgadvanced=, use_acout=off, use_bcout_sgadvanced=, use_bcout=off, use_pcout_sgadvanced=, use_pcout=off, use_multsignout_sgadvanced=, use_multsignout=off, use_carrycascout_sgadvanced=, use_carrycascout=off, pipeline_a_sgadvanced=, pipeline_a=1, pipeline_b_sgadvanced=, pipeline_b=1, pipeline_acout_sgadvanced=, pipeline_acout=1, pipeline_bcout_sgadvanced=, pipeline_bcout=1, pipeline_c_sgadvanced=, pipeline_c=on, pipeline_p_sgadvanced=, pipeline_p=on, pipeline_mult_sgadvanced=, pipeline_mult=on, pipeline_opmode_sgadvanced=, pipeline_opmode=on, pipeline_alumode_sgadvanced=, pipeline_alumode=on, pipeline_carryin_sgadvanced=, pipeline_carryin=on, pipeline_carryinsel_sgadvanced=, pipeline_carryinsel=on, rst_a_sgadvanced=, rst_a=off, rst_b_sgadvanced=, rst_b=off, rst_c_sgadvanced=, rst_c=off, rst_mult_sgadvanced=, rst_mult=off, rst_p_sgadvanced=, rst_p=off, rst_carry_in_sgadvanced=, rst_carry_in=off, rst_alumode_sgadvanced=, rst_alumode=off, rst_ctrl_sgadvanced=, rst_ctrl=off, en_a1_sgadvanced=, en_a1=off, en_a2_sgadvanced=, en_a2=off, en_b1_sgadvanced=, en_b1=off, en_b2_sgadvanced=, en_b2=off, en_c_sgadvanced=, en_c=off, en_mult_sgadvanced=, en_mult=off, en_p_sgadvanced=, en_p=off, en_carry_in_sgadvanced=, en_carry_in=off, en_alumode_sgadvanced=, en_alumode=off, en_multcarryin_sgadvanced=, en_multcarryin=off, en_ctrl_sgadvanced=, en_ctrl=off, use_synth_model_sgadvanced=, use_synth_model=off, addsub_mode_sgadvanced=, addsub_mode=ONE48, xl_useadderonly_sgadvanced=, xl_useadderonly=off, xl_use_area_sgadvanced=, xl_use_area=off, xl_area=[0,0,0,0,0,0,0], has_advanced_control=0, sggui_pos=-1,-1,-1,-1, block_type=dsp48e, block_version=, sg_icon_stat=75,136,6,1,white,blue,0,253a264c,right,,[ ],[ ], sg_mask_display=|, sg_list_contents=, sg_blockgui_xml=}
      mask sg_mask_display=|
      | fprintf('','COMMENT: begin icon graphics');
      | patch([0 75 75 0 0 ],[0 0 136 136 0 ],[0.77 0.82 0.91 ]);
      | plot([0 75 75 0 0 ],[0 0 136 136 0 ]);
      | patch([14.75 29.2 39.2 49.2 59.2 39.2 24.75 14.75 ],[79.1 79.1 89.1 79.1 89.1 89.1 89.1 79.1 ],[1 1 1 ]);
      | patch([24.75 39.2 29.2 14.75 24.75 ],[69.1 69.1 79.1 79.1 69.1 ],[0.931 0.946 0.973 ]);
      | patch([14.75 29.2 39.2 24.75 14.75 ],[59.1 59.1 69.1 69.1 59.1 ],[1 1 1 ]);
      | patch([24.75 59.2 49.2 39.2 29.2 14.75 24.75 ],[49.1 49.1 59.1 49.1 59.1 59.1 49.1 ],[0.931 0.946 0.973 ]);
      | fprintf('','COMMENT: end icon graphics');
      | fprintf('','COMMENT: begin icon text');
      | color('black');port_label('input',1,'a');
      | color('black');port_label('input',2,'b');
      | color('black');port_label('input',3,'opmode');
      | color('black');port_label('input',4,'alumode');
      | color('black');port_label('input',5,'carryin');
      | color('black');port_label('input',6,'carryinsel');
      | color('black');port_label('output',1,'p');
      | fprintf('','COMMENT: end icon text');
      mask prompts: use_a_sgadvanced ""; use_a "<tt>A</tt> or <tt>ACIN</tt> input"; use_b_sgadvanced ""; use_b "<tt>B</tt> or <tt>BCIN</tt> input"; reset_preg_sgadvanced ""; reset_preg "Reset <tt>p</tt> register on pattern detection"; pattern_from_creg_sgadvanced ""; pattern_from_creg "Pattern Input"; pattern "Pattern attribute"; mask_from_creg_sgadvanced ""; mask_from_creg "Mask Input"; pattern_mask "Mask attribute"; sel_rounding_mask_sgadvanced ""; sel_rounding_mask "Select rounding mask"; use_op_sgadvanced ""; use_op "Consolidate control port (<tt>opmode</tt>, <tt>alumode</tt>, <tt>carry_in</tt>, <tt>carry_in_sel</tt>)"; use_creg_sgadvanced ""; use_creg "Provide <tt>c</tt> port"; rst_all_sgadvanced ""; rst_all "Provide global reset port"; en_all_sgadvanced ""; en_all "Provide global enable port"; use_pcin_sgadvanced ""; use_pcin "Provide <tt>pcin</tt> port"; use_carrycascin_sgadvanced ""; use_carrycascin "Provide carry cascade in port"; use_multsignin_sgadvanced ""; use_multsignin "Provide multiplier sign cascade in port"; use_carryout_sgadvanced ""; use_carryout "Provide carry out port"; use_patterndetect_sgadvanced ""; use_patterndetect "Provide pattern detect port"; use_patternbdetect_sgadvanced ""; use_patternbdetect "Provide pattern bar detect port"; use_overflow_sgadvanced ""; use_overflow "Provide <tt>overflow</tt> port"; use_underflow_sgadvanced ""; use_underflow "Provide <tt>underflow</tt> port"; use_acout_sgadvanced ""; use_acout "Provide <tt>acout</tt> port"; use_bcout_sgadvanced ""; use_bcout "Provide <tt>bcout</tt> port"; use_pcout_sgadvanced ""; use_pcout "Provide <tt>pcout</tt> port"; use_multsignout_sgadvanced ""; use_multsignout "Provide multiplier sign cascade out port"; use_carrycascout_sgadvanced ""; use_carrycascout "Provide carry cascade out port"; pipeline_a_sgadvanced ""; pipeline_a "Length of <tt>a</tt>/<tt>acin</tt> pipeline"; pipeline_b_sgadvanced ""; pipeline_b "Length of <tt>b</tt>/<tt>bcin</tt> pipeline"; pipeline_acout_sgadvanced ""; pipeline_acout "Length of <tt>acout</tt> pipeline"; pipeline_bcout_sgadvanced ""; pipeline_bcout "Length of <tt>bcout</tt> pipeline"; pipeline_c_sgadvanced ""; pipeline_c "Pipeline <tt>c</tt>"; pipeline_p_sgadvanced ""; pipeline_p "Pipeline <tt>p</tt>"; pipeline_mult_sgadvanced ""; pipeline_mult "Pipeline multiplier"; pipeline_opmode_sgadvanced ""; pipeline_opmode "Pipeline <tt>opmode</tt>"; pipeline_alumode_sgadvanced ""; pipeline_alumode "Pipeline <tt>alumode</tt>"; pipeline_carryin_sgadvanced ""; pipeline_carryin "Pipeline carry in"; pipeline_carryinsel_sgadvanced ""; pipeline_carryinsel "Pipeline carry in select"; rst_a_sgadvanced ""; rst_a "Reset port for <tt>a</tt>/<tt>acin</tt>"; rst_b_sgadvanced ""; rst_b "Reset port for <tt>b</tt>/<tt>bcin</tt>"; rst_c_sgadvanced ""; rst_c "Reset port for <tt>c</tt>"; rst_mult_sgadvanced ""; rst_mult "Reset port for multiplier"; rst_p_sgadvanced ""; rst_p "Reset port for <tt>p</tt>"; rst_carry_in_sgadvanced ""; rst_carry_in "Reset port for carry in"; rst_alumode_sgadvanced ""; rst_alumode "Reset port for <tt>alumode</tt>"; rst_ctrl_sgadvanced ""; rst_ctrl "Reset port for controls<br> (<tt>opmode</tt> and <tt>carry_in_sel</tt>)"; en_a1_sgadvanced ""; en_a1 "Enable port for first <tt>a</tt>/<tt>acin</tt> register"; en_a2_sgadvanced ""; en_a2 "Enable port for second <tt>a</tt>/<tt>acin</tt> register"; en_b1_sgadvanced ""; en_b1 "Enable port for first <tt>b</tt>/<tt>bcin</tt> register"; en_b2_sgadvanced ""; en_b2 "Enable port for second <tt>b</tt>/<tt>bcin</tt> register"; en_c_sgadvanced ""; en_c "Enable port for <tt>c</tt>"; en_mult_sgadvanced ""; en_mult "Enable port for multiplier"; en_p_sgadvanced ""; en_p "Enable port for <tt>p<tt>"; en_carry_in_sgadvanced ""; en_carry_in "Enable port for carry in"; en_alumode_sgadvanced ""; en_alumode "Enable port for <tt>alumode<tt>"; en_multcarryin_sgadvanced ""; en_multcarryin "Enable port for multiplier carry in"; en_ctrl_sgadvanced ""; en_ctrl "Enable port for controls<br> (<tt>opmode</tt> and <tt>carry_in_sel</tt>)"; use_synth_model_sgadvanced ""; use_synth_model "Use synthesizable model"; addsub_mode_sgadvanced ""; addsub_mode "Mode of operation for the adder/subtractor"; xl_useadderonly_sgadvanced ""; xl_useadderonly "Use adder only"; xl_use_area_sgadvanced ""; xl_use_area "Define FPGA area for resource estimation"; xl_area "FPGA area [slices, FFs, BRAMs, LUTs, IOBs, emb. mults, TBUFs]"; has_advanced_control ""; sggui_pos ""; block_type ""; block_version ""; sg_icon_stat ""; sg_mask_display ""; sg_list_contents ""; sg_blockgui_xml ""
      mask help: Xilinx DSP48E
      mask init:
      | try
      |   tmp_gcb = gcb;
      |   tmp_gcbh = gcbh;
      |   if (strcmp('SysGenIndex',get_param(bdroot(tmp_gcbh),'tag')) && ~isempty(regexp(bdroot(tmp_gcb), '^xbs', 'once')))
      |     return;
      |   end;
      |   xlMungeMaskParams;
      |   block_config = 'sysgen_blockset:DSP48E_config';
      | 
      |   block_type='dsp48e';
      | 
      |   serialized_declarations = '{''addsub_mode''=>''Int'',''en_a1''=>''Bool'',''en_a2''=>''Bool'',''en_all''=>''Int'',''en_alumode''=>''Bool'',''en_b1''=>''Bool'',''en_b2''=>''Bool'',''en_c''=>''Bool'',''en_carry_in''=>''Bool'',''en_ctrl''=>''Bool'',''en_mult''=>''Bool'',''en_multcarryin''=>''Bool'',''en_p''=>''Bool'',''mask_from_creg''=>''Int'',''pattern''=>''String'',''pattern_from_creg''=>''Int'',''pattern_mask''=>''String'',''pipeline_a''=>''Int'',''pipeline_acout''=>''Int'',''pipeline_alumode''=>''Int'',''pipeline_b''=>''Int'',''pipeline_bcout''=>''Int'',''pipeline_c''=>''Int'',''pipeline_carryin''=>''Int'',''pipeline_carryinsel''=>''Int'',''pipeline_mult''=>''Bool'',''pipeline_opmode''=>''Int'',''pipeline_p''=>''Int'',''reset_preg''=>''Int'',''rst_a''=>''Int'',''rst_all''=>''Int'',''rst_alumode''=>''Int'',''rst_b''=>''Int'',''rst_c''=>''Int'',''rst_carry_in''=>''Int'',''rst_ctrl''=>''Int'',''rst_mult''=>''Int'',''rst_p''=>''Int'',''sel_rounding_mask''=>''Int'',''use_a''=>''Int'',''use_acout''=>''Int'',''use_b''=>''Int'',''use_bcout''=>''Int'',''use_carrycascin''=>''Int'',''use_carrycascout''=>''Int'',''use_carryout''=>''Bool'',''use_creg''=>''Int'',''use_multsignin''=>''Int'',''use_multsignout''=>''Int'',''use_op''=>''Int'',''use_overflow''=>''Bool'',''use_patternbdetect''=>''Bool'',''use_patterndetect''=>''Bool'',''use_pcin''=>''Int'',''use_pcout''=>''Int'',''use_synth_model''=>''Int'',''use_underflow''=>''Bool'',''xl_useadderonly''=>''Int'',''block_type''=>''String''}';
      |   ptable_ = xlblockprep(get_param(tmp_gcb, 'MaskWSVariables'));
      |   try
      |     xlBlockMoveCallback(tmp_gcbh);
      |   catch 
      |      clear global xl_updateicon_recursion_guard;
      |   end;
      | catch
      |   global dbgsysgen;
      |   if(~isempty(dbgsysgen) && dbgsysgen)
      |     e = regexprep(lasterr, '\n', '\nError: ');
      |     disp(['Error: While running MaskInit code on block ' tmp_gcb ': ' e]);
      |     error(e);
      |   end
      | end
      settings: CopyFcn=xlBlockMoveCallback(gcbh);  DeleteFcn=xlDestroyGui(gcbh);  ModelCloseFcn=xlDestroyGui(gcbh);  PreSaveFcn=xlBlockPreSaveCallback(gcbh);  PostSaveFcn=xlBlockPostSaveCallback(gcbh);  DestroyFcn=xlDestroyGui(gcbh);  OpenFcn=xlOpenGui(gcbh, 'dsp48e_gui.xml', @dsp48e_enablement, -1)  CloseFcn=xlDestroyGui(gcbh);  MoveFcn=xlBlockMoveCallback(gcbh);
      mask Help: eval('');xlDoc('-book','sysgen','-topic','DSP48E');
      mask StyleString: edit,popup(Direct from A Port|Cascaded from ACIN Port),edit,popup(Direct from B Port|Cascaded from BCIN Port),edit,checkbox,edit,popup(on|off),edit,edit,popup(on|off),edit,edit,popup(Select mask|Mode1|Mode2),edit,checkbox,edit,checkbox,edit,checkbox,edit,checkbox,edit,checkbox,edit,checkbox,edit,checkbox,edit,checkbox,edit,checkbox,edit,checkbox,edit,checkbox,edit,checkbox,edit,checkbox,edit,checkbox,edit,checkbox,edit,checkbox,edit,checkbox,edit,popup(0|1|2),edit,popup(0|1|2),edit,popup(0|1|2),edit,popup(0|1|2),edit,checkbox,edit,checkbox,edit,checkbox,edit,checkbox,edit,checkbox,edit,checkbox,edit,checkbox,edit,checkbox,edit,checkbox,edit,checkbox,edit,checkbox,edit,checkbox,edit,checkbox,edit,checkbox,edit,checkbox,edit,checkbox,edit,checkbox,edit,checkbox,edit,checkbox,edit,checkbox,edit,checkbox,edit,checkbox,edit,checkbox,edit,checkbox,edit,checkbox,edit,checkbox,edit,checkbox,edit,popup(ONE48|TWO24|FOUR12),edit,checkbox,edit,checkbox,edit,edit,edit,edit,edit,edit,edit,edit,edit
      mask Display:
      | fprintf('','COMMENT: begin icon graphics');
      | patch([0 75 75 0 0 ],[0 0 136 136 0 ],[0.77 0.82 0.91 ]);
      | plot([0 75 75 0 0 ],[0 0 136 136 0 ]);
      | patch([14.75 29.2 39.2 49.2 59.2 39.2 24.75 14.75 ],[79.1 79.1 89.1 79.1 89.1 89.1 89.1 79.1 ],[1 1 1 ]);
      | patch([24.75 39.2 29.2 14.75 24.75 ],[69.1 69.1 79.1 79.1 69.1 ],[0.931 0.946 0.973 ]);
      | patch([14.75 29.2 39.2 24.75 14.75 ],[59.1 59.1 69.1 69.1 59.1 ],[1 1 1 ]);
      | patch([24.75 59.2 49.2 39.2 29.2 14.75 24.75 ],[49.1 49.1 59.1 49.1 59.1 59.1 49.1 ],[0.931 0.946 0.973 ]);
      | fprintf('','COMMENT: end icon graphics');
      | fprintf('','COMMENT: begin icon text');
      | color('black');port_label('input',1,'a');
      | color('black');port_label('input',2,'b');
      | color('black');port_label('input',3,'opmode');
      | color('black');port_label('input',4,'alumode');
      | color('black');port_label('input',5,'carryin');
      | color('black');port_label('input',6,'carryinsel');
      | color('black');port_label('output',1,'p');
      | fprintf('','COMMENT: end icon text');
  "DSP48E1 " : S-Function  LoadFcn=xlBlockLoadCallback(gcbh);  FunctionName=sysgen  Parameters=ptable_  EnableBusSupport=off  mask(Xilinx DSP48E1 Block){use_a_sgadvanced=, use_a=Direct from A Port, use_b_sgadvanced=, use_b=Direct from B Port, addsub_mode_sgadvanced=, addsub_mode=ONE48, xl_useadderonly_sgadvanced=, xl_useadderonly=off, xl_dynamicmult_sgadvanced=, xl_dynamicmult=off, enable_preadder_sgadvanced=, enable_preadder=off, reset_preg_sgadvanced=, reset_preg=off, pattern_from_creg_sgadvanced=, pattern_from_creg=1, pattern='000000000000', mask_from_creg_sgadvanced=, mask_from_creg=1, pattern_mask='000000000000', use_op_sgadvanced=, use_op=off, use_creg_sgadvanced=, use_creg=off, rst_all_sgadvanced=, rst_all=off, en_all_sgadvanced=, en_all=off, use_pcin_sgadvanced=, use_pcin=off, use_carrycascin_sgadvanced=, use_carrycascin=off, use_multsignin_sgadvanced=, use_multsignin=off, use_carryout_sgadvanced=, use_carryout=off, use_patterndetect_sgadvanced=, use_patterndetect=off, use_patternbdetect_sgadvanced=, use_patternbdetect=off, use_overflow_sgadvanced=, use_overflow=off, use_underflow_sgadvanced=, use_underflow=off, use_acout_sgadvanced=, use_acout=off, use_bcout_sgadvanced=, use_bcout=off, use_pcout_sgadvanced=, use_pcout=off, use_multsignout_sgadvanced=, use_multsignout=off, use_carrycascout_sgadvanced=, use_carrycascout=off, pipeline_a_sgadvanced=, pipeline_a=1, pipeline_b_sgadvanced=, pipeline_b=1, pipeline_acout_sgadvanced=, pipeline_acout=1, pipeline_bcout_sgadvanced=, pipeline_bcout=1, pipeline_c_sgadvanced=, pipeline_c=on, pipeline_p_sgadvanced=, pipeline_p=on, pipeline_mult_sgadvanced=, pipeline_mult=on, pipeline_opmode_sgadvanced=, pipeline_opmode=on, pipeline_alumode_sgadvanced=, pipeline_alumode=on, pipeline_carryin_sgadvanced=, pipeline_carryin=on, pipeline_carryinsel_sgadvanced=, pipeline_carryinsel=on, dreg_sgadvanced=, dreg=off, adreg_sgadvanced=, adreg=off, register_inmode_sgadvanced=, register_inmode=off, rst_a_sgadvanced=, rst_a=off, rst_b_sgadvanced=, rst_b=off, rst_c_sgadvanced=, rst_c=off, rst_mult_sgadvanced=, rst_mult=off, rst_p_sgadvanced=, rst_p=off, rst_carry_in_sgadvanced=, rst_carry_in=off, rst_alumode_sgadvanced=, rst_alumode=off, rst_ctrl_sgadvanced=, rst_ctrl=off, reset_port_d_sgadvanced=, reset_port_d=off, reset_port_inmode_sgadvanced=, reset_port_inmode=off, en_a1_sgadvanced=, en_a1=off, en_a2_sgadvanced=, en_a2=off, en_b1_sgadvanced=, en_b1=off, en_b2_sgadvanced=, en_b2=off, en_c_sgadvanced=, en_c=off, en_mult_sgadvanced=, en_mult=off, en_p_sgadvanced=, en_p=off, en_carry_in_sgadvanced=, en_carry_in=off, en_alumode_sgadvanced=, en_alumode=off, en_multcarryin_sgadvanced=, en_multcarryin=off, en_ctrl_sgadvanced=, en_ctrl=off, enable_port_regd_sgadvanced=, enable_port_regd=off, enable_port_regad_sgadvanced=, enable_port_regad=off, enable_port_reginmode_sgadvanced=, enable_port_reginmode=off, use_synth_model_sgadvanced=, use_synth_model=off, xl_use_area_sgadvanced=, xl_use_area=off, xl_area=[0,0,0,0,0,0,0], has_advanced_control=0, sggui_pos=-1,-1,-1,-1, block_type=dsp48e1, block_version=, sg_icon_stat=75,136,6,1,white,blue,0,253a264c,right,,[ ],[ ], sg_mask_display=|, sg_list_contents=, sg_blockgui_xml=}
      mask sg_mask_display=|
      | fprintf('','COMMENT: begin icon graphics');
      | patch([0 75 75 0 0 ],[0 0 136 136 0 ],[0.77 0.82 0.91 ]);
      | plot([0 75 75 0 0 ],[0 0 136 136 0 ]);
      | patch([14.75 29.2 39.2 49.2 59.2 39.2 24.75 14.75 ],[79.1 79.1 89.1 79.1 89.1 89.1 89.1 79.1 ],[1 1 1 ]);
      | patch([24.75 39.2 29.2 14.75 24.75 ],[69.1 69.1 79.1 79.1 69.1 ],[0.931 0.946 0.973 ]);
      | patch([14.75 29.2 39.2 24.75 14.75 ],[59.1 59.1 69.1 69.1 59.1 ],[1 1 1 ]);
      | patch([24.75 59.2 49.2 39.2 29.2 14.75 24.75 ],[49.1 49.1 59.1 49.1 59.1 59.1 49.1 ],[0.931 0.946 0.973 ]);
      | fprintf('','COMMENT: end icon graphics');
      | fprintf('','COMMENT: begin icon text');
      | color('black');port_label('input',1,'a');
      | color('black');port_label('input',2,'b');
      | color('black');port_label('input',3,'opmode');
      | color('black');port_label('input',4,'alumode');
      | color('black');port_label('input',5,'carryin');
      | color('black');port_label('input',6,'carryinsel');
      | color('black');port_label('output',1,'p');
      | fprintf('','COMMENT: end icon text');
      mask prompts: use_a_sgadvanced ""; use_a "<tt>A</tt> or <tt>ACIN</tt> input"; use_b_sgadvanced ""; use_b "<tt>B</tt> or <tt>BCIN</tt> input"; addsub_mode_sgadvanced ""; addsub_mode "SIMD Mode of Adder/Subtractor/Accumulator"; xl_useadderonly_sgadvanced ""; xl_useadderonly "Do not use multiplier"; xl_dynamicmult_sgadvanced ""; xl_dynamicmult "Use dynamic multiplier mode"; enable_preadder_sgadvanced ""; enable_preadder "Use preadder"; reset_preg_sgadvanced ""; reset_preg "Reset <tt>p</tt> register on pattern detection"; pattern_from_creg_sgadvanced ""; pattern_from_creg "Pattern Input"; pattern "Pattern attribute"; mask_from_creg_sgadvanced ""; mask_from_creg "Mask Input"; pattern_mask "Mask attribute"; use_op_sgadvanced ""; use_op "Consolidate control port (<tt>opmode</tt>, <tt>alumode</tt>, <tt>carry_in</tt>, <tt>carry_in_sel</tt>)"; use_creg_sgadvanced ""; use_creg "Provide <tt>c</tt> port"; rst_all_sgadvanced ""; rst_all "Provide global reset port"; en_all_sgadvanced ""; en_all "Provide global enable port"; use_pcin_sgadvanced ""; use_pcin "Provide <tt>pcin</tt> port"; use_carrycascin_sgadvanced ""; use_carrycascin "Provide carry cascade in port"; use_multsignin_sgadvanced ""; use_multsignin "Provide multiplier sign cascade in port"; use_carryout_sgadvanced ""; use_carryout "Provide carry out port"; use_patterndetect_sgadvanced ""; use_patterndetect "Provide pattern detect port"; use_patternbdetect_sgadvanced ""; use_patternbdetect "Provide pattern bar detect port"; use_overflow_sgadvanced ""; use_overflow "Provide <tt>overflow</tt> port"; use_underflow_sgadvanced ""; use_underflow "Provide <tt>underflow</tt> port"; use_acout_sgadvanced ""; use_acout "Provide <tt>acout</tt> port"; use_bcout_sgadvanced ""; use_bcout "Provide <tt>bcout</tt> port"; use_pcout_sgadvanced ""; use_pcout "Provide <tt>pcout</tt> port"; use_multsignout_sgadvanced ""; use_multsignout "Provide multiplier sign cascade out port"; use_carrycascout_sgadvanced ""; use_carrycascout "Provide carry cascade out port"; pipeline_a_sgadvanced ""; pipeline_a "Length of <tt>a</tt>/<tt>acin</tt> pipeline"; pipeline_b_sgadvanced ""; pipeline_b "Length of <tt>b</tt>/<tt>bcin</tt> pipeline"; pipeline_acout_sgadvanced ""; pipeline_acout "Length of <tt>acout</tt> pipeline"; pipeline_bcout_sgadvanced ""; pipeline_bcout "Length of <tt>bcout</tt> pipeline"; pipeline_c_sgadvanced ""; pipeline_c "Pipeline <tt>c</tt>"; pipeline_p_sgadvanced ""; pipeline_p "Pipeline <tt>p</tt>"; pipeline_mult_sgadvanced ""; pipeline_mult "Pipeline multiplier"; pipeline_opmode_sgadvanced ""; pipeline_opmode "Pipeline <tt>opmode</tt>"; pipeline_alumode_sgadvanced ""; pipeline_alumode "Pipeline <tt>alumode</tt>"; pipeline_carryin_sgadvanced ""; pipeline_carryin "Pipeline carry in"; pipeline_carryinsel_sgadvanced ""; pipeline_carryinsel "Pipeline carry in select"; dreg_sgadvanced ""; dreg "Pipeline preadder input register <tt>d</tt>"; adreg_sgadvanced ""; adreg "Pipeline preadder output register <tt>ad</tt>"; register_inmode_sgadvanced ""; register_inmode "Pipeline  <tt>INMODE</tt> register"; rst_a_sgadvanced ""; rst_a "Reset port for <tt>a</tt>/<tt>acin</tt>"; rst_b_sgadvanced ""; rst_b "Reset port for <tt>b</tt>/<tt>bcin</tt>"; rst_c_sgadvanced ""; rst_c "Reset port for <tt>c</tt>"; rst_mult_sgadvanced ""; rst_mult "Reset port for multiplier"; rst_p_sgadvanced ""; rst_p "Reset port for <tt>p</tt>"; rst_carry_in_sgadvanced ""; rst_carry_in "Reset port for carry in"; rst_alumode_sgadvanced ""; rst_alumode "Reset port for <tt>alumode</tt>"; rst_ctrl_sgadvanced ""; rst_ctrl "Reset port for controls<br> (<tt>opmode</tt> and <tt>carry_in_sel</tt>)"; reset_port_d_sgadvanced ""; reset_port_d "Reset port for <tt>d</tt> and <tt>ad</tt>"; reset_port_inmode_sgadvanced ""; reset_port_inmode "Reset port for <tt>INMODE</tt>"; en_a1_sgadvanced ""; en_a1 "Enable port for first <tt>a</tt>/<tt>acin</tt> register"; en_a2_sgadvanced ""; en_a2 "Enable port for second <tt>a</tt>/<tt>acin</tt> register"; en_b1_sgadvanced ""; en_b1 "Enable port for first <tt>b</tt>/<tt>bcin</tt> register"; en_b2_sgadvanced ""; en_b2 "Enable port for second <tt>b</tt>/<tt>bcin</tt> register"; en_c_sgadvanced ""; en_c "Enable port for <tt>c</tt>"; en_mult_sgadvanced ""; en_mult "Enable port for multiplier"; en_p_sgadvanced ""; en_p "Enable port for <tt>p<tt>"; en_carry_in_sgadvanced ""; en_carry_in "Enable port for carry in"; en_alumode_sgadvanced ""; en_alumode "Enable port for <tt>alumode<tt>"; en_multcarryin_sgadvanced ""; en_multcarryin "Enable port for multiplier carry in"; en_ctrl_sgadvanced ""; en_ctrl "Enable port for controls<br> (<tt>opmode</tt> and <tt>carry_in_sel</tt>)"; enable_port_regd_sgadvanced ""; enable_port_regd "Enable port for <tt>d</tt>"; enable_port_regad_sgadvanced ""; enable_port_regad "Enable port for <tt>ad</tt>"; enable_port_reginmode_sgadvanced ""; enable_port_reginmode "Enable port for <tt>INMODE</tt>"; use_synth_model_sgadvanced ""; use_synth_model "Use synthesizable model"; xl_use_area_sgadvanced ""; xl_use_area "Define FPGA area for resource estimation"; xl_area "FPGA area [slices, FFs, BRAMs, LUTs, IOBs, emb. mults, TBUFs]"; has_advanced_control ""; sggui_pos ""; block_type ""; block_version ""; sg_icon_stat ""; sg_mask_display ""; sg_list_contents ""; sg_blockgui_xml ""
      mask help: Xilinx DSP48E1
      mask init:
      | try
      |   tmp_gcb = gcb;
      |   tmp_gcbh = gcbh;
      |   if (strcmp('SysGenIndex',get_param(bdroot(tmp_gcbh),'tag')) && ~isempty(regexp(bdroot(tmp_gcb), '^xbs', 'once')))
      |     return;
      |   end;
      |   xlMungeMaskParams;
      |   block_config = 'sysgen_blockset:DSP48E1_config';
      | 
      |   block_type='dsp48e1';
      | 
      |   serialized_declarations = '{''addsub_mode''=>''Int'',''adreg''=>''Bool'',''dreg''=>''Bool'',''en_a1''=>''Bool'',''en_a2''=>''Bool'',''en_all''=>''Int'',''en_alumode''=>''Bool'',''en_b1''=>''Bool'',''en_b2''=>''Bool'',''en_c''=>''Bool'',''en_carry_in''=>''Bool'',''en_ctrl''=>''Bool'',''en_mult''=>''Bool'',''en_multcarryin''=>''Bool'',''en_p''=>''Bool'',''enable_port_regad''=>''Bool'',''enable_port_regd''=>''Bool'',''enable_port_reginmode''=>''Bool'',''enable_preadder''=>''Bool'',''mask_from_creg''=>''Int'',''pattern''=>''String'',''pattern_from_creg''=>''Int'',''pattern_mask''=>''String'',''pipeline_a''=>''Int'',''pipeline_acout''=>''Int'',''pipeline_alumode''=>''Int'',''pipeline_b''=>''Int'',''pipeline_bcout''=>''Int'',''pipeline_c''=>''Int'',''pipeline_carryin''=>''Int'',''pipeline_carryinsel''=>''Int'',''pipeline_mult''=>''Bool'',''pipeline_opmode''=>''Int'',''pipeline_p''=>''Int'',''register_inmode''=>''Bool'',''reset_port_d''=>''Int'',''reset_port_inmode''=>''Int'',''reset_preg''=>''Int'',''rst_a''=>''Int'',''rst_all''=>''Int'',''rst_alumode''=>''Int'',''rst_b''=>''Int'',''rst_c''=>''Int'',''rst_carry_in''=>''Int'',''rst_ctrl''=>''Int'',''rst_mult''=>''Int'',''rst_p''=>''Int'',''use_a''=>''Int'',''use_acout''=>''Int'',''use_b''=>''Int'',''use_bcout''=>''Int'',''use_carrycascin''=>''Int'',''use_carrycascout''=>''Int'',''use_carryout''=>''Bool'',''use_creg''=>''Int'',''use_multsignin''=>''Int'',''use_multsignout''=>''Int'',''use_op''=>''Int'',''use_overflow''=>''Bool'',''use_patternbdetect''=>''Bool'',''use_patterndetect''=>''Bool'',''use_pcin''=>''Int'',''use_pcout''=>''Int'',''use_synth_model''=>''Int'',''use_underflow''=>''Bool'',''xl_dynamicmult''=>''Int'',''xl_useadderonly''=>''Int'',''block_type''=>''String''}';
      |   ptable_ = xlblockprep(get_param(tmp_gcb, 'MaskWSVariables'));
      |   try
      |     xlBlockMoveCallback(tmp_gcbh);
      |   catch 
      |      clear global xl_updateicon_recursion_guard;
      |   end;
      | catch
      |   global dbgsysgen;
      |   if(~isempty(dbgsysgen) && dbgsysgen)
      |     e = regexprep(lasterr, '\n', '\nError: ');
      |     disp(['Error: While running MaskInit code on block ' tmp_gcb ': ' e]);
      |     error(e);
      |   end
      | end
      settings: CopyFcn=xlBlockMoveCallback(gcbh);  DeleteFcn=xlDestroyGui(gcbh);  ModelCloseFcn=xlDestroyGui(gcbh);  PreSaveFcn=xlBlockPreSaveCallback(gcbh);  PostSaveFcn=xlBlockPostSaveCallback(gcbh);  DestroyFcn=xlDestroyGui(gcbh);  OpenFcn=xlOpenGui(gcbh, 'dsp48e1_gui.xml', @dsp48e1_enablement, -1)  CloseFcn=xlDestroyGui(gcbh);  MoveFcn=xlBlockMoveCallback(gcbh);
      mask Help: eval('');xlDoc('-book','sysgen','-topic','DSP48E1');
      mask StyleString: edit,popup(Direct from A Port|Cascaded from ACIN Port),edit,popup(Direct from B Port|Cascaded from BCIN Port),edit,popup(ONE48|TWO24|FOUR12),edit,checkbox,edit,checkbox,edit,checkbox,edit,checkbox,edit,popup(1|2),edit,edit,popup(1|2|3|4),edit,edit,checkbox,edit,checkbox,edit,checkbox,edit,checkbox,edit,checkbox,edit,checkbox,edit,checkbox,edit,checkbox,edit,checkbox,edit,checkbox,edit,checkbox,edit,checkbox,edit,checkbox,edit,checkbox,edit,checkbox,edit,checkbox,edit,checkbox,edit,popup(0|1|2),edit,popup(0|1|2),edit,popup(0|1|2),edit,popup(0|1|2),edit,checkbox,edit,checkbox,edit,checkbox,edit,checkbox,edit,checkbox,edit,checkbox,edit,checkbox,edit,checkbox,edit,checkbox,edit,checkbox,edit,checkbox,edit,checkbox,edit,checkbox,edit,checkbox,edit,checkbox,edit,checkbox,edit,checkbox,edit,checkbox,edit,checkbox,edit,checkbox,edit,checkbox,edit,checkbox,edit,checkbox,edit,checkbox,edit,checkbox,edit,checkbox,edit,checkbox,edit,checkbox,edit,checkbox,edit,checkbox,edit,checkbox,edit,checkbox,edit,checkbox,edit,checkbox,edit,checkbox,edit,checkbox,edit,edit,edit,edit,edit,edit,edit,edit,edit
      mask Display:
      | fprintf('','COMMENT: begin icon graphics');
      | patch([0 75 75 0 0 ],[0 0 136 136 0 ],[0.77 0.82 0.91 ]);
      | plot([0 75 75 0 0 ],[0 0 136 136 0 ]);
      | patch([14.75 29.2 39.2 49.2 59.2 39.2 24.75 14.75 ],[79.1 79.1 89.1 79.1 89.1 89.1 89.1 79.1 ],[1 1 1 ]);
      | patch([24.75 39.2 29.2 14.75 24.75 ],[69.1 69.1 79.1 79.1 69.1 ],[0.931 0.946 0.973 ]);
      | patch([14.75 29.2 39.2 24.75 14.75 ],[59.1 59.1 69.1 69.1 59.1 ],[1 1 1 ]);
      | patch([24.75 59.2 49.2 39.2 29.2 14.75 24.75 ],[49.1 49.1 59.1 49.1 59.1 59.1 49.1 ],[0.931 0.946 0.973 ]);
      | fprintf('','COMMENT: end icon graphics');
      | fprintf('','COMMENT: begin icon text');
      | color('black');port_label('input',1,'a');
      | color('black');port_label('input',2,'b');
      | color('black');port_label('input',3,'opmode');
      | color('black');port_label('input',4,'alumode');
      | color('black');port_label('input',5,'carryin');
      | color('black');port_label('input',6,'carryinsel');
      | color('black');port_label('output',1,'p');
      | fprintf('','COMMENT: end icon text');
  Delay : S-Function  LoadFcn=xlBlockLoadCallback(gcbh);  FunctionName=sysgen  Parameters=ptable_  EnableBusSupport=off  mask(Xilinx Delay Block){infoedit=Hardware notes: A delay line is a chain, each link of which is an SRL16 followed by a flip-flop., rst_sgadvanced=, rst=off, infoeditControl=Selection of Reset will increase slice count due to use of real FFs and instead of SRLs, en_sgadvanced=, en=off, latency=1, dbl_ovrd_sgadvanced=, dbl_ovrd=off, reg_retiming_sgadvanced=, reg_retiming=off, xl_use_area_sgadvanced=, xl_use_area=off, xl_area=[0,0,0,0,0,0,0], has_advanced_control=0, sggui_pos=-1,-1,-1,-1, block_type=delay, block_version=, sg_icon_stat=60,56,1,1,white,blue,0,07b98262,right,,[ ],[ ], sg_mask_display=|, sg_list_contents=, sg_blockgui_xml=}
      mask sg_mask_display=|
      | fprintf('','COMMENT: begin icon graphics');
      | patch([0 60 60 0 0 ],[0 0 56 56 0 ],[0.77 0.82 0.91 ]);
      | plot([0 60 60 0 0 ],[0 0 56 56 0 ]);
      | patch([12.2 23.76 31.76 39.76 47.76 31.76 20.2 12.2 ],[36.88 36.88 44.88 36.88 44.88 44.88 44.88 36.88 ],[1 1 1 ]);
      | patch([20.2 31.76 23.76 12.2 20.2 ],[28.88 28.88 36.88 36.88 28.88 ],[0.931 0.946 0.973 ]);
      | patch([12.2 23.76 31.76 20.2 12.2 ],[20.88 20.88 28.88 28.88 20.88 ],[1 1 1 ]);
      | patch([20.2 47.76 39.76 31.76 23.76 12.2 20.2 ],[12.88 12.88 20.88 12.88 20.88 20.88 12.88 ],[0.931 0.946 0.973 ]);
      | fprintf('','COMMENT: end icon graphics');
      | fprintf('','COMMENT: begin icon text');
      |
      |
      | color('black');disp('z^{-1}','texmode','on');
      | fprintf('','COMMENT: end icon text');
      mask prompts: infoedit ""; rst_sgadvanced ""; rst "Provide synchronous reset port"; infoeditControl ""; en_sgadvanced ""; en "Provide enable port"; dbl_ovrd_sgadvanced ""; dbl_ovrd "Override with doubles"; reg_retiming_sgadvanced ""; reg_retiming "Implement using behavioral HDL."; xl_use_area_sgadvanced ""; xl_use_area "Define FPGA area for resource estimation"; xl_area "FPGA area [slices, FFs, BRAMs, LUTs, IOBs, emb. mults, TBUFs]"; has_advanced_control ""; sggui_pos ""; block_type ""; block_version ""; sg_icon_stat ""; sg_mask_display ""; sg_list_contents ""; sg_blockgui_xml ""
      mask help: Hardware notes: A delay line is a chain, each link of which is an SRL16 followed by a flip-flop.
      mask init:
      | try
      |   tmp_gcb = gcb;
      |   tmp_gcbh = gcbh;
      |   if (strcmp('SysGenIndex',get_param(bdroot(tmp_gcbh),'tag')) && ~isempty(regexp(bdroot(tmp_gcb), '^xbs', 'once')))
      |     return;
      |   end;
      |   xlMungeMaskParams;
      |   block_config = 'sysgen_blockset:Delay_config';
      | 
      |   block_type='delay';
      | 
      |   serialized_declarations = '{''dbl_ovrd''=>''Int'',''en''=>''Int'',''latency''=>''Int'',''reg_retiming''=>''Int'',''rst''=>''Int'',''block_type''=>''String''}';
      |   ptable_ = xlblockprep(get_param(tmp_gcb, 'MaskWSVariables'));
      |   try
      |     xlBlockMoveCallback(tmp_gcbh);
      |   catch 
      |      clear global xl_updateicon_recursion_guard;
      |   end;
      | catch
      |   global dbgsysgen;
      |   if(~isempty(dbgsysgen) && dbgsysgen)
      |     e = regexprep(lasterr, '\n', '\nError: ');
      |     disp(['Error: While running MaskInit code on block ' tmp_gcb ': ' e]);
      |     error(e);
      |   end
      | end
      settings: CopyFcn=xlBlockMoveCallback(gcbh);  DeleteFcn=xlDestroyGui(gcbh);  ModelCloseFcn=xlDestroyGui(gcbh);  PreSaveFcn=xlBlockPreSaveCallback(gcbh);  PostSaveFcn=xlBlockPostSaveCallback(gcbh);  DestroyFcn=xlDestroyGui(gcbh);  OpenFcn=xlOpenGui(gcbh, 'delay_gui.xml', @xlmagicenablement, -1)  CloseFcn=xlDestroyGui(gcbh);  MoveFcn=xlBlockMoveCallback(gcbh);
      mask Help: eval('');xlDoc('-book','sysgen','-topic','Delay');
      mask Display:
      | fprintf('','COMMENT: begin icon graphics');
      | patch([0 60 60 0 0 ],[0 0 56 56 0 ],[0.77 0.82 0.91 ]);
      | plot([0 60 60 0 0 ],[0 0 56 56 0 ]);
      | patch([12.2 23.76 31.76 39.76 47.76 31.76 20.2 12.2 ],[36.88 36.88 44.88 36.88 44.88 44.88 44.88 36.88 ],[1 1 1 ]);
      | patch([20.2 31.76 23.76 12.2 20.2 ],[28.88 28.88 36.88 36.88 28.88 ],[0.931 0.946 0.973 ]);
      | patch([12.2 23.76 31.76 20.2 12.2 ],[20.88 20.88 28.88 28.88 20.88 ],[1 1 1 ]);
      | patch([20.2 47.76 39.76 31.76 23.76 12.2 20.2 ],[12.88 12.88 20.88 12.88 20.88 20.88 12.88 ],[0.931 0.946 0.973 ]);
      | fprintf('','COMMENT: end icon graphics');
      | fprintf('','COMMENT: begin icon text');
      | 
      | 
      | color('black');disp('z^{-1}','texmode','on');
      | fprintf('','COMMENT: end icon text');
  Depuncture : S-Function  LoadFcn=xlBlockLoadCallback(gcbh);  FunctionName=sysgen  Parameters=ptable_  EnableBusSupport=off  mask(Xilinx Depuncturer Block){infoedit=Depunctures convolutional codes.  Reads values from the input port, inserts symbols at the locations specified by zeros in the puncture code, and presents the results at the output port. <br><br>Hardware notes: In hardware this block costs nothing., insert_char=[1 0 0], insert_string='100', dbl_ovrd_sgadvanced=, dbl_ovrd=off, has_advanced_control=0, sggui_pos=-1,-1,-1,-1, block_type=insert, block_version=, sg_icon_stat=65,32,1,1,white,blue,0,e3c99253,right,,[ ],[ ], sg_mask_display=|, sg_list_contents=, sg_blockgui_xml=}
      mask sg_mask_display=|
      | fprintf('','COMMENT: begin icon graphics');
      | patch([0 65 65 0 0 ],[0 0 32 32 0 ],[0.77 0.82 0.91 ]);
      | plot([0 65 65 0 0 ],[0 0 32 32 0 ]);
      | patch([23.1 28.88 32.88 36.88 40.88 32.88 27.1 23.1 ],[20.44 20.44 24.44 20.44 24.44 24.44 24.44 20.44 ],[1 1 1 ]);
      | patch([27.1 32.88 28.88 23.1 27.1 ],[16.44 16.44 20.44 20.44 16.44 ],[0.931 0.946 0.973 ]);
      | patch([23.1 28.88 32.88 27.1 23.1 ],[12.44 12.44 16.44 16.44 12.44 ],[1 1 1 ]);
      | patch([27.1 40.88 36.88 32.88 28.88 23.1 27.1 ],[8.44 8.44 12.44 8.44 12.44 12.44 8.44 ],[0.931 0.946 0.973 ]);
      | fprintf('','COMMENT: end icon graphics');
      | fprintf('','COMMENT: begin icon text');
      |
      |
      | color('black');disp('Depuncture');
      | fprintf('','COMMENT: end icon text');
      mask prompts: infoedit ""; insert_char "Depuncture code"; insert_string "Symbol to insert"; dbl_ovrd_sgadvanced ""; dbl_ovrd "Override with doubles"; has_advanced_control ""; sggui_pos ""; block_type ""; block_version ""; sg_icon_stat ""; sg_mask_display ""; sg_list_contents ""; sg_blockgui_xml ""
      mask help:
      | Depunctures convolutional codes.  Reads values from the input port, inserts symbols at the locations specified by zeros in the puncture code, and presents the results at the output port.
      |
      | Hardware notes: In hardware this block costs nothing.
      mask init:
      | try
      |   tmp_gcb = gcb;
      |   tmp_gcbh = gcbh;
      |   if (strcmp('SysGenIndex',get_param(bdroot(tmp_gcbh),'tag')) && ~isempty(regexp(bdroot(tmp_gcb), '^xbs', 'once')))
      |     return;
      |   end;
      |   xlMungeMaskParams;
      |   block_config = 'sysgen_blockset:Depuncture_config';
      | 
      |   block_type='insert';
      | 
      |   serialized_declarations = '{''insert_char''=>''IntVector'',''insert_code''=>''String'',''insert_int''=>''Int'',''insert_string''=>''String'',''string_int''=>''Int'',''block_type''=>''String''}';
      |   ptable_ = xlblockprep(get_param(tmp_gcb, 'MaskWSVariables'));
      |   try
      |     xlBlockMoveCallback(tmp_gcbh);
      |   catch 
      |      clear global xl_updateicon_recursion_guard;
      |   end;
      | catch
      |   global dbgsysgen;
      |   if(~isempty(dbgsysgen) && dbgsysgen)
      |     e = regexprep(lasterr, '\n', '\nError: ');
      |     disp(['Error: While running MaskInit code on block ' tmp_gcb ': ' e]);
      |     error(e);
      |   end
      | end
      settings: CopyFcn=xlBlockMoveCallback(gcbh);  DeleteFcn=xlDestroyGui(gcbh);  ModelCloseFcn=xlDestroyGui(gcbh);  PreSaveFcn=xlBlockPreSaveCallback(gcbh);  PostSaveFcn=xlBlockPostSaveCallback(gcbh);  DestroyFcn=xlDestroyGui(gcbh);  OpenFcn=xlOpenGui(gcbh, 'depuncture_gui.xml', @xlmagicenablement, -1)  CloseFcn=xlDestroyGui(gcbh);  MoveFcn=xlBlockMoveCallback(gcbh);
      mask Help: eval('');xlDoc('-book','sysgen','-topic','Depuncture');
      mask Display:
      | fprintf('','COMMENT: begin icon graphics');
      | patch([0 65 65 0 0 ],[0 0 32 32 0 ],[0.77 0.82 0.91 ]);
      | plot([0 65 65 0 0 ],[0 0 32 32 0 ]);
      | patch([23.1 28.88 32.88 36.88 40.88 32.88 27.1 23.1 ],[20.44 20.44 24.44 20.44 24.44 24.44 24.44 20.44 ],[1 1 1 ]);
      | patch([27.1 32.88 28.88 23.1 27.1 ],[16.44 16.44 20.44 20.44 16.44 ],[0.931 0.946 0.973 ]);
      | patch([23.1 28.88 32.88 27.1 23.1 ],[12.44 12.44 16.44 16.44 12.44 ],[1 1 1 ]);
      | patch([27.1 40.88 36.88 32.88 28.88 23.1 27.1 ],[8.44 8.44 12.44 8.44 12.44 12.44 8.44 ],[0.931 0.946 0.973 ]);
      | fprintf('','COMMENT: end icon graphics');
      | fprintf('','COMMENT: begin icon text');
      | 
      | 
      | color('black');disp('Depuncture');
      | fprintf('','COMMENT: end icon text');
  Disregard Subsystem : S-Function  Tag=discardX  LoadFcn=xlBlockLoadCallback(gcbh);  FunctionName=xlpermissive  Parameters=''  EnableBusSupport=off  mask(Xilinx Disregard Subsystem For Generation Block){infoedit=Place this block into a subsystem to have System Generator ignore the subsystem during code generation. This block can be used in combination with the Simulation Multiplexer block to provide an alternative simulation model for another subsystem (e.g., to provide a simulation model for a black box)., ShowPortLabels=, has_advanced_control=0, sggui_pos=-1,-1,-1,-1, block_type=disregard, block_version=, sg_icon_stat=58,58,-1,-1,darkgray,black,0,07734,right,,[ ],[ ], sg_mask_display=|, sg_list_contents=, sg_blockgui_xml=}
      mask sg_mask_display=|
      | fprintf('','COMMENT: begin icon graphics');
      | patch([0 58 58 0 0 ],[0 0 58 58 0 ],[0.1 0.1 0.1 ]);
      | plot([0 58 58 0 0 ],[0 0 58 58 0 ]);
      | patch([11.2 22.76 30.76 38.76 46.76 30.76 19.2 11.2 ],[37.88 37.88 45.88 37.88 45.88 45.88 45.88 37.88 ],[0.33 0.33 0.33 ]);
      | patch([19.2 30.76 22.76 11.2 19.2 ],[29.88 29.88 37.88 37.88 29.88 ],[0.261 0.261 0.261 ]);
      | patch([11.2 22.76 30.76 19.2 11.2 ],[21.88 21.88 29.88 29.88 21.88 ],[0.33 0.33 0.33 ]);
      | patch([19.2 46.76 38.76 30.76 22.76 11.2 19.2 ],[13.88 13.88 21.88 13.88 21.88 21.88 13.88 ],[0.261 0.261 0.261 ]);
      | fprintf('','COMMENT: end icon graphics');
      | fprintf('','COMMENT: begin icon text');
      | fprintf('','COMMENT: end icon text');
      mask prompts: infoedit ""; ShowPortLabels ""; has_advanced_control ""; sggui_pos ""; block_type ""; block_version ""; sg_icon_stat ""; sg_mask_display ""; sg_list_contents ""; sg_blockgui_xml ""
      mask help: Place this block into a subsystem to have System Generator ignore the subsystem during code generation. This block can be used in combination with the Simulation Multiplexer block to provide an alternative simulation model for another subsystem (e.g., to provide a simulation model for a black box).
      mask init:
      | try
      |   tmp_gcb = gcb;
      |   tmp_gcbh = gcbh;
      |   if (strcmp('SysGenIndex',get_param(bdroot(tmp_gcbh),'tag')) && ~isempty(regexp(bdroot(tmp_gcb), '^xbs', 'once')))
      |     return;
      |   end;
      |   xlMungeMaskParams;
      | 
      |   block_type='disregard';
      | 
      |   serialized_declarations = '{''block_type''=>''String''}';
      |   xldisregard_init();
      |   ptable_ = xlblockprep(get_param(tmp_gcb, 'MaskWSVariables'));
      |   try
      |     xlBlockMoveCallback(tmp_gcbh);
      |   catch 
      |      clear global xl_updateicon_recursion_guard;
      |   end;
      | catch
      |   global dbgsysgen;
      |   if(~isempty(dbgsysgen) && dbgsysgen)
      |     e = regexprep(lasterr, '\n', '\nError: ');
      |     disp(['Error: While running MaskInit code on block ' tmp_gcb ': ' e]);
      |     error(e);
      |   end
      | end
      settings: AttributesFormatString=Disregard Subsystem\nFor Generation  CopyFcn=xlBlockMoveCallback(gcbh);  DeleteFcn=xlDestroyGui(gcbh);  ModelCloseFcn=xlDestroyGui(gcbh);  PreSaveFcn=xlBlockPreSaveCallback(gcbh);  PostSaveFcn=xlBlockPostSaveCallback(gcbh);  DestroyFcn=xlDestroyGui(gcbh);  OpenFcn=xlOpenGui(gcbh, 'disregard_gui.xml', -1, -1)  CloseFcn=xlDestroyGui(gcbh);  MoveFcn=xlBlockMoveCallback(gcbh);
      mask Help: eval('');xlDoc('-book','sysgen','-topic','Disregard_Subsystem');
      mask Display:
      | fprintf('','COMMENT: begin icon graphics');
      | patch([0 58 58 0 0 ],[0 0 58 58 0 ],[0.1 0.1 0.1 ]);
      | plot([0 58 58 0 0 ],[0 0 58 58 0 ]);
      | patch([11.2 22.76 30.76 38.76 46.76 30.76 19.2 11.2 ],[37.88 37.88 45.88 37.88 45.88 45.88 45.88 37.88 ],[0.33 0.33 0.33 ]);
      | patch([19.2 30.76 22.76 11.2 19.2 ],[29.88 29.88 37.88 37.88 29.88 ],[0.261 0.261 0.261 ]);
      | patch([11.2 22.76 30.76 19.2 11.2 ],[21.88 21.88 29.88 29.88 21.88 ],[0.33 0.33 0.33 ]);
      | patch([19.2 46.76 38.76 30.76 22.76 11.2 19.2 ],[13.88 13.88 21.88 13.88 21.88 21.88 13.88 ],[0.261 0.261 0.261 ]);
      | fprintf('','COMMENT: end icon graphics');
      | fprintf('','COMMENT: begin icon text');
      | fprintf('','COMMENT: end icon text');
  Divide : S-Function  LoadFcn=xlBlockLoadCallback(gcbh);  FunctionName=sysgen  Parameters=ptable_  EnableBusSupport=off  mask(Xilinx Divider Block){infoedit=Blocking: Wait for data on all inputs, allow back-pressure.<br>NonBlocking: operate every cycle in which all inputs are valid, no back-pressure., flow_control=NonBlocking, axi_optimize_goal=Resources, algorithm_type=High_Radix, infoedit1=Specify output fraction-width for Fixed-point division., fractional_width=16, latency=0, rate=1, has_a_tlast=off, has_a_tuser=off, has_b_tlast=off, has_b_tuser=off, en=off, has_result_tready=off, result_tlast_behv_sgadvanced=, result_tlast_behv=Pass_A_TLAST, has_underflow=off, has_overflow=off, has_invalid_op=off, has_divide_by_zero=off, xl_use_area_sgadvanced=, xl_use_area=off, xl_area=[0,0,0,0,0,0,0], fpo_op_type=mergeddivide, has_advanced_control=0, sggui_pos=-1,-1,-1,-1, block_type=divide, block_version=, sg_icon_stat=55,55,2,1,white,blue,0,857da21d,right,,[ ],[ ], sg_mask_display=|, sg_list_contents=, sg_blockgui_xml=}
      mask sg_mask_display=|
      | fprintf('','COMMENT: begin icon graphics');
      | patch([0 55 55 0 0 ],[0 0 55 55 0 ],[0.77 0.82 0.91 ]);
      | plot([0 55 55 0 0 ],[0 0 55 55 0 ]);
      | patch([11.425 21.54 28.54 35.54 42.54 28.54 18.425 11.425 ],[34.77 34.77 41.77 34.77 41.77 41.77 41.77 34.77 ],[1 1 1 ]);
      | patch([18.425 28.54 21.54 11.425 18.425 ],[27.77 27.77 34.77 34.77 27.77 ],[0.931 0.946 0.973 ]);
      | patch([11.425 21.54 28.54 18.425 11.425 ],[20.77 20.77 27.77 27.77 20.77 ],[1 1 1 ]);
      | patch([18.425 42.54 35.54 28.54 21.54 11.425 18.425 ],[13.77 13.77 20.77 13.77 20.77 20.77 13.77 ],[0.931 0.946 0.973 ]);
      | fprintf('','COMMENT: end icon graphics');
      | fprintf('','COMMENT: begin icon text');
      | color('black');port_label('input',1,'a');
      | color('black');port_label('input',2,'b');
      | color('black');port_label('output',1,'op');
      | fprintf('','COMMENT: end icon text');
      mask prompts: infoedit ""; flow_control "Flow Control"; axi_optimize_goal "Optimize Goal"; algorithm_type "Algorithm Type"; infoedit1 ""; fractional_width "Output Fractional width"; rate "Cycles/operation"; has_a_tlast "Has TLAST"; has_a_tuser "Has TUSER"; has_b_tlast "Has TLAST"; has_b_tuser "Has TUSER"; en "Provide enable port"; has_result_tready "Has Result TREADY"; result_tlast_behv_sgadvanced ""; result_tlast_behv "Output TLAST behavior"; has_underflow "UNDERFLOW"; has_overflow "OVERFLOW"; has_invalid_op "INVALID_OP"; has_divide_by_zero "DIVIDE_BY_ZERO"; xl_use_area_sgadvanced ""; xl_use_area "Define FPGA area for resource estimation"; xl_area "FPGA area [slices, FFs, BRAMs, LUTs, IOBs, emb. mults, TBUFs]"; fpo_op_type ""; has_advanced_control ""; sggui_pos ""; block_type ""; block_version ""; sg_icon_stat ""; sg_mask_display ""; sg_list_contents ""; sg_blockgui_xml ""
      mask help:
      | Blocking: Wait for data on all inputs, allow back-pressure.
      | NonBlocking: operate every cycle in which all inputs are valid, no back-pressure.
      mask init:
      | try
      |   tmp_gcb = gcb;
      |   tmp_gcbh = gcbh;
      |   if (strcmp('SysGenIndex',get_param(bdroot(tmp_gcbh),'tag')) && ~isempty(regexp(bdroot(tmp_gcb), '^xbs', 'once')))
      |     return;
      |   end;
      |   xlMungeMaskParams;
      |   block_config = 'sysgen:FPOBlockDescriptor_config';
      | 
      |   block_type='divide';
      | 
      |   serialized_declarations = '{''algorithm_type''=>''String'',''axi_optimize_goal''=>''String'',''en''=>''Bool'',''flow_control''=>''String'',''fpo_op_type''=>''String'',''fractional_width''=>''Int'',''has_a_tlast''=>''Bool'',''has_a_tuser''=>''Bool'',''has_b_tlast''=>''Bool'',''has_b_tuser''=>''Bool'',''has_divide_by_zero''=>''Bool'',''has_invalid_op''=>''Bool'',''has_overflow''=>''Bool'',''has_result_tready''=>''Bool'',''has_underflow''=>''Bool'',''latency''=>''Int'',''rate''=>''Int'',''result_tlast_behv''=>''Int'',''block_type''=>''String''}';
      |   ptable_ = xlblockprep(get_param(tmp_gcb, 'MaskWSVariables'));
      |   try
      |     xlBlockMoveCallback(tmp_gcbh);
      |   catch 
      |      clear global xl_updateicon_recursion_guard;
      |   end;
      | catch
      |   global dbgsysgen;
      |   if(~isempty(dbgsysgen) && dbgsysgen)
      |     e = regexprep(lasterr, '\n', '\nError: ');
      |     disp(['Error: While running MaskInit code on block ' tmp_gcb ': ' e]);
      |     error(e);
      |   end
      | end
      settings: CopyFcn=xlBlockMoveCallback(gcbh);  DeleteFcn=xlDestroyGui(gcbh);  ModelCloseFcn=xlDestroyGui(gcbh);  PreSaveFcn=xlBlockPreSaveCallback(gcbh);  PostSaveFcn=xlBlockPostSaveCallback(gcbh);  DestroyFcn=xlDestroyGui(gcbh);  OpenFcn=xlOpenGui(gcbh, 'divide_gui.xml', @divideenablement, @divideaction)  CloseFcn=xlDestroyGui(gcbh);  MoveFcn=xlBlockMoveCallback(gcbh);
      mask Help: eval('');xlDoc('-book','sysgen','-topic','Divide');
      mask StyleString: edit,popup(Blocking|NonBlocking),popup(Resources|Performance),popup(Radix2|High_Radix),edit,edit,edit,edit,checkbox,checkbox,checkbox,checkbox,checkbox,checkbox,edit,popup(Pass_A_TLAST|Pass_B_TLAST|OR_all_TLASTs|AND_all_TLASTs),checkbox,checkbox,checkbox,checkbox,edit,checkbox,edit,edit,edit,edit,edit,edit,edit,edit,edit,edit
      mask Display:
      | fprintf('','COMMENT: begin icon graphics');
      | patch([0 55 55 0 0 ],[0 0 55 55 0 ],[0.77 0.82 0.91 ]);
      | plot([0 55 55 0 0 ],[0 0 55 55 0 ]);
      | patch([11.425 21.54 28.54 35.54 42.54 28.54 18.425 11.425 ],[34.77 34.77 41.77 34.77 41.77 41.77 41.77 34.77 ],[1 1 1 ]);
      | patch([18.425 28.54 21.54 11.425 18.425 ],[27.77 27.77 34.77 34.77 27.77 ],[0.931 0.946 0.973 ]);
      | patch([11.425 21.54 28.54 18.425 11.425 ],[20.77 20.77 27.77 27.77 20.77 ],[1 1 1 ]);
      | patch([18.425 42.54 35.54 28.54 21.54 11.425 18.425 ],[13.77 13.77 20.77 13.77 20.77 20.77 13.77 ],[0.931 0.946 0.973 ]);
      | fprintf('','COMMENT: end icon graphics');
      | fprintf('','COMMENT: begin icon text');
      | color('black');port_label('input',1,'a');
      | color('black');port_label('input',2,'b');
      | color('black');port_label('output',1,'op');
      | fprintf('','COMMENT: end icon text');
  "Divider Generator 2.0 " : S-Function  LoadFcn=xlBlockLoadCallback(gcbh);  FunctionName=sysgen  Parameters=ptable_  EnableBusSupport=off  mask(Xilinx Divider Generator 2.0 Block){dividend_and_quotient_width=2, divisor_width=32, algorithm_type=Radix2, remainder_type=Remainder, fractional_width=16, clocks_per_division=1, divide_by_zero_detect=off, latency_configuration=Automatic, latency=25, en=off, rst=off, xl_use_area=off, xl_area=[0,0,0,0,0,0,0], ip_name=Divider Generator, ip_version=2.0, dsptool_ready=true, wrapper_available=true, ce=1, sclr=1, sclr_ce_priority=SCLR_overrides_CE, operand_sign=Signed, port_translation_map={ 'ce' => 'en', 'sclr' => 'rst' }, ipcore_fpga_part=xlipgetpartsetting(gcb, {'virtex4', 'xc4vsx35', '-10', 'ff668'}), has_advanced_control=0, sggui_pos=-1,-1,-1,-1, block_type=div_gen_v2_0, block_version=, sg_icon_stat=95,142,-1,-1,white,blue,0,07734,right,,[ ],[ ], sg_mask_display=|, sg_list_contents=, sg_blockgui_xml=}
      mask sg_mask_display=|
      | fprintf('','COMMENT: begin icon graphics');
      | patch([0 95 95 0 0 ],[0 0 142 142 0 ],[0.77 0.82 0.91 ]);
      | plot([0 95 95 0 0 ],[0 0 142 142 0 ]);
      | patch([18.075 36.86 49.86 62.86 75.86 49.86 31.075 18.075 ],[85.43 85.43 98.43 85.43 98.43 98.43 98.43 85.43 ],[1 1 1 ]);
      | patch([31.075 49.86 36.86 18.075 31.075 ],[72.43 72.43 85.43 85.43 72.43 ],[0.931 0.946 0.973 ]);
      | patch([18.075 36.86 49.86 31.075 18.075 ],[59.43 59.43 72.43 72.43 59.43 ],[1 1 1 ]);
      | patch([31.075 75.86 62.86 49.86 36.86 18.075 31.075 ],[46.43 46.43 59.43 46.43 59.43 59.43 46.43 ],[0.931 0.946 0.973 ]);
      | fprintf('','COMMENT: end icon graphics');
      | fprintf('','COMMENT: begin icon text');
      | fprintf('','COMMENT: end icon text');
      mask prompts: dividend_and_quotient_width "Dividend and quotient width"; divisor_width "Divisor width"; algorithm_type "Algorithm Type"; remainder_type "Remainder type"; fractional_width "Fractional width"; clocks_per_division "Clocks per division"; divide_by_zero_detect "Detect divide by zero"; latency_configuration "Latency configuration"; xl_use_area "Define FPGA area for resource estimation"; xl_area "FPGA area [slices, FFs, BRAMs, LUTs, IOBs, emb. mults, TBUFs]"; ip_name ""; ip_version ""; dsptool_ready ""; wrapper_available ""; ce ""; sclr ""; sclr_ce_priority ""; operand_sign ""; port_translation_map ""; ipcore_fpga_part ""; has_advanced_control ""; sggui_pos ""; block_type ""; block_version ""; sg_icon_stat ""; sg_mask_display ""; sg_list_contents ""; sg_blockgui_xml ""
      mask help: Xilinx Divider Generator 2.0
      mask init:
      | try
      |   tmp_gcb = gcb;
      |   tmp_gcbh = gcbh;
      |   if (strcmp('SysGenIndex',get_param(bdroot(tmp_gcbh),'tag')) && ~isempty(regexp(bdroot(tmp_gcb), '^xbs', 'once')))
      |     return;
      |   end;
      |   xlMungeMaskParams;
      |   block_config = 'sysgen_blockset:Removed_config';
      | 
      |   block_type='div_gen_v2_0';
      | nport = get_param(gcbh, 'ports');
      | nin = nport(1);
      | nout = nport(2);
      | 
      |   serialized_declarations = '{''algorithm_type''=>''String'',''ce''=>''Bool'',''clocks_per_division''=>''String'',''divide_by_zero_detect''=>''Bool'',''dividend_and_quotient_width''=>''Int'',''divisor_width''=>''Int'',''dsptool_ready''=>''Bool'',''en''=>''Bool'',''fractional_width''=>''Int'',''ip_name''=>''String'',''ip_version''=>''String'',''ipcore_fpga_part''=>''StringVector'',''latency''=>''Int'',''latency_configuration''=>''String'',''operand_sign''=>''String'',''port_translation_map''=>''String'',''remainder_type''=>''String'',''rst''=>''Bool'',''sclr''=>''Bool'',''sclr_ce_priority''=>''String'',''wrapper_available''=>''Bool'',''xl_use_area''=>''Bool'',''block_type''=>''String'',''nin''=>''Double'',''nout''=>''Double''}';
      |   xldivider_generator_v2_0_init();
      |   ptable_ = xlblockprep(get_param(tmp_gcb, 'MaskWSVariables'));
      |   try
      |     xlBlockMoveCallback(tmp_gcbh);
      |   catch 
      |      clear global xl_updateicon_recursion_guard;
      |   end;
      | catch
      |   global dbgsysgen;
      |   if(~isempty(dbgsysgen) && dbgsysgen)
      |     e = regexprep(lasterr, '\n', '\nError: ');
      |     disp(['Error: While running MaskInit code on block ' tmp_gcb ': ' e]);
      |     error(e);
      |   end
      | end
      settings: CopyFcn=xlBlockMoveCallback(gcbh);  DeleteFcn=xlDestroyGui(gcbh);  ModelCloseFcn=xlDestroyGui(gcbh);  PreSaveFcn=xlBlockPreSaveCallback(gcbh);  PostSaveFcn=xlBlockPostSaveCallback(gcbh);  DestroyFcn=xlDestroyGui(gcbh);  OpenFcn=xlOpenGui(gcbh, 'div_gen_v2_0_gui.xml', @xlremovedenablement, -1)  CloseFcn=xlDestroyGui(gcbh);  MoveFcn=xlBlockMoveCallback(gcbh);
      mask Help: eval('');xlDoc('-book','sysgen','-topic','Divider_Generator_2_0');
      mask StyleString: edit,edit,popup(Radix2|High_Radix),popup(Remainder|Fractional),edit,popup(1|2|4|8),checkbox,popup(Automatic|Manual),edit,checkbox,checkbox,checkbox,edit,edit,edit,edit,edit,edit,edit,edit,edit,edit,edit,edit,edit,edit,edit,edit,edit,edit,edit
      mask Display:
      | fprintf('','COMMENT: begin icon graphics');
      | patch([0 95 95 0 0 ],[0 0 142 142 0 ],[0.77 0.82 0.91 ]);
      | plot([0 95 95 0 0 ],[0 0 142 142 0 ]);
      | patch([18.075 36.86 49.86 62.86 75.86 49.86 31.075 18.075 ],[85.43 85.43 98.43 85.43 98.43 98.43 98.43 85.43 ],[1 1 1 ]);
      | patch([31.075 49.86 36.86 18.075 31.075 ],[72.43 72.43 85.43 85.43 72.43 ],[0.931 0.946 0.973 ]);
      | patch([18.075 36.86 49.86 31.075 18.075 ],[59.43 59.43 72.43 72.43 59.43 ],[1 1 1 ]);
      | patch([31.075 75.86 62.86 49.86 36.86 18.075 31.075 ],[46.43 46.43 59.43 46.43 59.43 59.43 46.43 ],[0.931 0.946 0.973 ]);
      | fprintf('','COMMENT: end icon graphics');
      | fprintf('','COMMENT: begin icon text');
      | fprintf('','COMMENT: end icon text');
  "Divider Generator 3.0 " : S-Function  LoadFcn=xlBlockLoadCallback(gcbh);  FunctionName=sysgen  Parameters=ptable_  EnableBusSupport=off  mask(Xilinx Divider Generator 3.0 Block){dividend_and_quotient_width=2, divisor_width=32, algorithm_type=Radix2, remainder_type=Remainder, fractional_width=16, clocks_per_division=1, divide_by_zero_detect=off, latency_configuration=Automatic, latency=25, ce=off, sclr=off, xl_use_area=off, xl_area=[0,0,0,0,0,0,0], sclr_ce_priority=CE_overrides_SCLR, operand_sign=Signed, ip_name=Divider Generator, ip_version=3.0, dsptool_ready=true, wrapper_available=true, port_translation_map={ 'ce' => 'en', 'sclr' => 'rst' }, ipcore_fpga_part=xlipgetpartsetting(gcb, {'virtex4', 'xc4vsx35', '-10', 'ff668'}), ipcore_verbose=false, has_advanced_control=0, sggui_pos=-1,-1,-1,-1, block_type=div_gen_v3_0, block_version=, sg_icon_stat=95,142,2,3,white,blue,0,1fc55160,right,,[ ],[ ], sg_mask_display=|, sg_list_contents=, sg_blockgui_xml=}
      mask sg_mask_display=|
      | fprintf('','COMMENT: begin icon graphics');
      | patch([0 95 95 0 0 ],[0 0 142 142 0 ],[0.77 0.82 0.91 ]);
      | plot([0 95 95 0 0 ],[0 0 142 142 0 ]);
      | patch([18.075 36.86 49.86 62.86 75.86 49.86 31.075 18.075 ],[85.43 85.43 98.43 85.43 98.43 98.43 98.43 85.43 ],[1 1 1 ]);
      | patch([31.075 49.86 36.86 18.075 31.075 ],[72.43 72.43 85.43 85.43 72.43 ],[0.931 0.946 0.973 ]);
      | patch([18.075 36.86 49.86 31.075 18.075 ],[59.43 59.43 72.43 72.43 59.43 ],[1 1 1 ]);
      | patch([31.075 75.86 62.86 49.86 36.86 18.075 31.075 ],[46.43 46.43 59.43 46.43 59.43 59.43 46.43 ],[0.931 0.946 0.973 ]);
      | fprintf('','COMMENT: end icon graphics');
      | fprintf('','COMMENT: begin icon text');
      | color('black');port_label('input',1,'dividend');
      | color('black');port_label('input',2,'divisor');
      | color('black');port_label('output',1,'rfd');
      | color('black');port_label('output',2,'quotient');
      | color('black');port_label('output',3,'fractional');
      | fprintf('','COMMENT: end icon text');
      mask prompts: dividend_and_quotient_width "Dividend and quotient width"; divisor_width "Divisor width"; algorithm_type "Algorithm Type"; remainder_type "Remainder type"; fractional_width "Fractional width"; clocks_per_division "Clocks per division"; divide_by_zero_detect "Detect divide by zero"; latency_configuration "Latency configuration"; ce "en"; sclr "rst"; xl_use_area "Define FPGA area for resource estimation"; xl_area "FPGA area [slices, FFs, BRAMs, LUTs, IOBs, emb. mults, TBUFs]"; sclr_ce_priority ""; operand_sign ""; ip_name ""; ip_version ""; dsptool_ready ""; wrapper_available ""; port_translation_map ""; ipcore_fpga_part ""; ipcore_verbose ""; has_advanced_control ""; sggui_pos ""; block_type ""; block_version ""; sg_icon_stat ""; sg_mask_display ""; sg_list_contents ""; sg_blockgui_xml ""
      mask help: Xilinx Divider Generator 3.0
      mask init:
      | try
      |   tmp_gcb = gcb;
      |   tmp_gcbh = gcbh;
      |   if (strcmp('SysGenIndex',get_param(bdroot(tmp_gcbh),'tag')) && ~isempty(regexp(bdroot(tmp_gcb), '^xbs', 'once')))
      |     return;
      |   end;
      |   xlMungeMaskParams;
      |   block_config = 'sysgen:coregenimport_config';
      | 
      |   block_type='div_gen_v3_0';
      | 
      |   serialized_declarations = '{''algorithm_type''=>''String'',''ce''=>''Bool'',''clocks_per_division''=>''String'',''divide_by_zero_detect''=>''Bool'',''dividend_and_quotient_width''=>''Int'',''divisor_width''=>''Int'',''dsptool_ready''=>''Bool'',''fractional_width''=>''Int'',''ip_name''=>''String'',''ip_version''=>''String'',''ipcore_fpga_part''=>''StringVector'',''ipcore_verbose''=>''Bool'',''latency''=>''Int'',''latency_configuration''=>''String'',''operand_sign''=>''String'',''port_translation_map''=>''String'',''remainder_type''=>''String'',''sclr''=>''Bool'',''sclr_ce_priority''=>''String'',''wrapper_available''=>''Bool'',''xl_use_area''=>''Bool'',''block_type''=>''String''}';
      |   ptable_ = xlblockprep(get_param(tmp_gcb, 'MaskWSVariables'));
      |   try
      |     xlBlockMoveCallback(tmp_gcbh);
      |   catch 
      |      clear global xl_updateicon_recursion_guard;
      |   end;
      | catch
      |   global dbgsysgen;
      |   if(~isempty(dbgsysgen) && dbgsysgen)
      |     e = regexprep(lasterr, '\n', '\nError: ');
      |     disp(['Error: While running MaskInit code on block ' tmp_gcb ': ' e]);
      |     error(e);
      |   end
      | end
      settings: CopyFcn=xlBlockMoveCallback(gcbh);  DeleteFcn=xlDestroyGui(gcbh);  ModelCloseFcn=xlDestroyGui(gcbh);  PreSaveFcn=xlBlockPreSaveCallback(gcbh);  PostSaveFcn=xlBlockPostSaveCallback(gcbh);  DestroyFcn=xlDestroyGui(gcbh);  OpenFcn=xlOpenGui(gcbh, 'div_gen_v3_0_gui.xml', @xlipmagiccallback, @xlipmagicaction)  CloseFcn=xlDestroyGui(gcbh);  MoveFcn=xlBlockMoveCallback(gcbh);
      mask Help: eval('');xlDoc('-book','sysgen','-topic','Divider_Generator_3_0');
      mask StyleString: edit,edit,popup(Radix2|High_Radix),popup(Remainder|Fractional),edit,popup(1|2|4|8),checkbox,popup(Automatic|Manual),edit,checkbox,checkbox,checkbox,edit,edit,edit,edit,edit,edit,edit,edit,edit,edit,edit,edit,edit,edit,edit,edit,edit,edit
      mask Display:
      | fprintf('','COMMENT: begin icon graphics');
      | patch([0 95 95 0 0 ],[0 0 142 142 0 ],[0.77 0.82 0.91 ]);
      | plot([0 95 95 0 0 ],[0 0 142 142 0 ]);
      | patch([18.075 36.86 49.86 62.86 75.86 49.86 31.075 18.075 ],[85.43 85.43 98.43 85.43 98.43 98.43 98.43 85.43 ],[1 1 1 ]);
      | patch([31.075 49.86 36.86 18.075 31.075 ],[72.43 72.43 85.43 85.43 72.43 ],[0.931 0.946 0.973 ]);
      | patch([18.075 36.86 49.86 31.075 18.075 ],[59.43 59.43 72.43 72.43 59.43 ],[1 1 1 ]);
      | patch([31.075 75.86 62.86 49.86 36.86 18.075 31.075 ],[46.43 46.43 59.43 46.43 59.43 59.43 46.43 ],[0.931 0.946 0.973 ]);
      | fprintf('','COMMENT: end icon graphics');
      | fprintf('','COMMENT: begin icon text');
      | color('black');port_label('input',1,'dividend');
      | color('black');port_label('input',2,'divisor');
      | color('black');port_label('output',1,'rfd');
      | color('black');port_label('output',2,'quotient');
      | color('black');port_label('output',3,'fractional');
      | fprintf('','COMMENT: end icon text');
  "Divider Generator 4.0 " : S-Function  LoadFcn=xlBlockLoadCallback(gcbh);  FunctionName=sysgen  Parameters=ptable_  EnableBusSupport=off  mask(Xilinx Divider Generator 4.0 Block){infoedit=Divider Generator 4.0, algorithm_type=Radix2, remainder_type=Remainder, fractional_width=16, clocks_per_division=1, divide_by_zero_detect=off, flowcontrol=NonBlocking, optimizegoal=Resources, latency_configuration=Automatic, latency=20, dividend_has_tuser=off, dividend_has_tlast=off, divisor_has_tuser=off, divisor_has_tlast=off, aclken=off, aresetn=off, outtready=off, outtlastbehv=Null, trim_axipin_name=on, xl_use_area=off, xl_area=[0,0,0,0,0,0,0], dividend_tuser_width=1, divisor_tuser_width=1, operand_sign=Signed, dividend_and_quotient_width=16, divisor_width=16, ip_name=Divider Generator, ip_version=4.0, dsptool_ready=true, ipcore_usecache=true, ipcore_useipmodelcache=true, wrapper_available=true, port_translation_map={'aclken' => 'en','aresetn' => 'rst'}, ipcore_fpga_part=xlipgetpartsetting(gcb, {'virtex7', 'xc7v1500t', '-2', 'fhg1157'}), ipcore_verbose=false, has_advanced_control=0, sggui_pos=-1,-1,-1,-1, block_type=div_gen_v4_0, block_version=, sg_icon_stat=95,143,4,3,white,blue,0,3f82dac1,right,,[2 2 3 3 ],[4 4 4 ], sg_mask_display=|, sg_list_contents=, sg_blockgui_xml=}
      mask sg_mask_display=|
      | fprintf('','COMMENT: begin icon graphics');
      | patch([0 0 2 2 ],[136 77 77 136 ],[6.025000e-001 6.400000e-001 7.075000e-001 ]);
      | patch([0 0 2 2 ],[66 7 7 66 ],[4.350000e-001 4.600000e-001 5.050000e-001 ]);
      | patch([93 93 95 95 ],[130 8 8 130 ],[2.675000e-001 2.800000e-001 3.025000e-001 ]);
      | patch([2 92 92 2 2 ],[0 0 143 143 0 ],[7.700000e-001 8.200000e-001 9.100000e-001 ]);
      | plot([2 92 92 2 2 ],[0 0 143 143 0 ]);
      |
      |
      | patch([18.075 36.86 49.86 62.86 75.86 49.86 31.075 18.075 ],[85.43 85.43 98.43 85.43 98.43 98.43 98.43 85.43 ],[1 1 1 ]);
      | patch([31.075 49.86 36.86 18.075 31.075 ],[72.43 72.43 85.43 85.43 72.43 ],[0.931 0.946 0.973 ]);
      | patch([18.075 36.86 49.86 31.075 18.075 ],[59.43 59.43 72.43 72.43 59.43 ],[1 1 1 ]);
      | patch([31.075 75.86 62.86 49.86 36.86 18.075 31.075 ],[46.43 46.43 59.43 46.43 59.43 59.43 46.43 ],[0.931 0.946 0.973 ]);
      | fprintf('','COMMENT: end icon graphics');
      | fprintf('','COMMENT: begin icon text');
      | color('black');port_label('input',1,'  dividend_tvalid  ');
      | color('black');port_label('input',2,'  dividend_tdata_dividend  ');
      | color('black');port_label('input',3,'  divisor_tvalid  ');
      | color('black');port_label('input',4,'  divisor_tdata_divisor  ');
      | color('black');port_label('output',1,'  dout_tvalid  ');
      | color('black');port_label('output',2,'  dout_tdata_quotient  ');
      | color('black');port_label('output',3,'  dout_tdata_remainder  ');
      | fprintf('','COMMENT: end icon text');
      mask prompts: infoedit ""; algorithm_type "Algorithm Type"; remainder_type "Remainder Type"; fractional_width "Fractional width"; clocks_per_division "Radix2 throughput"; divide_by_zero_detect "Detect Divide-by-Zero"; flowcontrol "AXI behaviour"; optimizegoal "AXI implementation emphasis"; latency_configuration "Latency Configuration"; dividend_has_tuser "Has TUSER"; dividend_has_tlast "Has TLAST"; divisor_has_tuser "Has TUSER"; divisor_has_tlast "Has TLAST"; outtready "m_axis_dout_tready"; outtlastbehv "Input TLAST combination for output"; trim_axipin_name "Display shortened port names"; xl_use_area "Define FPGA area for resource estimation"; xl_area "FPGA area [slices, FFs, BRAMs, LUTs, IOBs, emb. mults, TBUFs]"; dividend_tuser_width ""; divisor_tuser_width ""; operand_sign ""; dividend_and_quotient_width ""; divisor_width ""; ip_name ""; ip_version ""; dsptool_ready ""; ipcore_usecache ""; ipcore_useipmodelcache ""; wrapper_available ""; port_translation_map ""; ipcore_fpga_part ""; ipcore_verbose ""; has_advanced_control ""; sggui_pos ""; block_type ""; block_version ""; sg_icon_stat ""; sg_mask_display ""; sg_list_contents ""; sg_blockgui_xml ""
      mask help: Divider Generator 4.0
      mask init:
      | try
      |   tmp_gcb = gcb;
      |   tmp_gcbh = gcbh;
      |   if (strcmp('SysGenIndex',get_param(bdroot(tmp_gcbh),'tag')) && ~isempty(regexp(bdroot(tmp_gcb), '^xbs', 'once')))
      |     return;
      |   end;
      |   xlMungeMaskParams;
      |   block_config = 'sysgen:coregenimport_config';
      | 
      |   block_type='div_gen_v4_0';
      | 
      |   serialized_declarations = '{''aclken''=>''Bool'',''algorithm_type''=>''String'',''aresetn''=>''Bool'',''clocks_per_division''=>''String'',''divide_by_zero_detect''=>''Bool'',''dividend_and_quotient_width''=>''Int'',''dividend_has_tlast''=>''Bool'',''dividend_has_tuser''=>''Bool'',''dividend_tuser_width''=>''Int'',''divisor_has_tlast''=>''Bool'',''divisor_has_tuser''=>''Bool'',''divisor_tuser_width''=>''Int'',''divisor_width''=>''Int'',''dsptool_ready''=>''Bool'',''flowcontrol''=>''String'',''fractional_width''=>''Int'',''ip_name''=>''String'',''ip_version''=>''String'',''ipcore_fpga_part''=>''StringVector'',''ipcore_usecache''=>''Bool'',''ipcore_useipmodelcache''=>''Bool'',''ipcore_verbose''=>''Bool'',''latency''=>''Int'',''latency_configuration''=>''String'',''operand_sign''=>''String'',''optimizegoal''=>''String'',''outtlastbehv''=>''String'',''outtready''=>''Bool'',''port_translation_map''=>''String'',''remainder_type''=>''String'',''trim_axipin_name''=>''Int'',''wrapper_available''=>''Bool'',''xl_use_area''=>''Bool'',''block_type''=>''String''}';
      |   ptable_ = xlblockprep(get_param(tmp_gcb, 'MaskWSVariables'));
      |   try
      |     xlBlockMoveCallback(tmp_gcbh);
      |   catch 
      |      clear global xl_updateicon_recursion_guard;
      |   end;
      | catch
      |   global dbgsysgen;
      |   if(~isempty(dbgsysgen) && dbgsysgen)
      |     e = regexprep(lasterr, '\n', '\nError: ');
      |     disp(['Error: While running MaskInit code on block ' tmp_gcb ': ' e]);
      |     error(e);
      |   end
      | end
      settings: CopyFcn=xlBlockMoveCallback(gcbh);  DeleteFcn=xlDestroyGui(gcbh);  ModelCloseFcn=xlDestroyGui(gcbh);  PreSaveFcn=xlBlockPreSaveCallback(gcbh);  PostSaveFcn=xlBlockPostSaveCallback(gcbh);  DestroyFcn=xlDestroyGui(gcbh);  OpenFcn=xlOpenGui(gcbh, 'div_gen_v4_0_gui.xml', @xlipmagiccallback, -1)  CloseFcn=xlDestroyGui(gcbh);  MoveFcn=xlBlockMoveCallback(gcbh);
      mask Help: eval('');xlDoc('-book','sysgen','-topic','Divider_Generator_4_0');
      mask StyleString: edit,popup(Radix2|High_Radix),popup(Remainder|Fractional),edit,popup(1|2|4|8),checkbox,popup(NonBlocking|Blocking),popup(Resources|Performance),popup(Automatic|Manual),edit,checkbox,checkbox,checkbox,checkbox,checkbox,checkbox,checkbox,popup(Null|Pass_Dividend_TLAST|Pass_Divisor_TLAST|OR_all_TLASTs|AND_all_TLASTs),checkbox,checkbox,edit,edit,edit,edit,edit,edit,edit,edit,edit,edit,edit,edit,edit,edit,edit,edit,edit,edit,edit,edit,edit,edit,edit
      mask Display:
      | fprintf('','COMMENT: begin icon graphics');
      | patch([0 0 2 2 ],[136 77 77 136 ],[6.025000e-001 6.400000e-001 7.075000e-001 ]);
      | patch([0 0 2 2 ],[66 7 7 66 ],[4.350000e-001 4.600000e-001 5.050000e-001 ]);
      | patch([93 93 95 95 ],[130 8 8 130 ],[2.675000e-001 2.800000e-001 3.025000e-001 ]);
      | patch([2 92 92 2 2 ],[0 0 143 143 0 ],[7.700000e-001 8.200000e-001 9.100000e-001 ]);
      | plot([2 92 92 2 2 ],[0 0 143 143 0 ]);
      | 
      | 
      | patch([18.075 36.86 49.86 62.86 75.86 49.86 31.075 18.075 ],[85.43 85.43 98.43 85.43 98.43 98.43 98.43 85.43 ],[1 1 1 ]);
      | patch([31.075 49.86 36.86 18.075 31.075 ],[72.43 72.43 85.43 85.43 72.43 ],[0.931 0.946 0.973 ]);
      | patch([18.075 36.86 49.86 31.075 18.075 ],[59.43 59.43 72.43 72.43 59.43 ],[1 1 1 ]);
      | patch([31.075 75.86 62.86 49.86 36.86 18.075 31.075 ],[46.43 46.43 59.43 46.43 59.43 59.43 46.43 ],[0.931 0.946 0.973 ]);
      | fprintf('','COMMENT: end icon graphics');
      | fprintf('','COMMENT: begin icon text');
      | color('black');port_label('input',1,'  dividend_tvalid  ');
      | color('black');port_label('input',2,'  dividend_tdata_dividend  ');
      | color('black');port_label('input',3,'  divisor_tvalid  ');
      | color('black');port_label('input',4,'  divisor_tdata_divisor  ');
      | color('black');port_label('output',1,'  dout_tvalid  ');
      | color('black');port_label('output',2,'  dout_tdata_quotient  ');
      | color('black');port_label('output',3,'  dout_tdata_remainder  ');
      | fprintf('','COMMENT: end icon text');
  Down Sample : S-Function  LoadFcn=xlBlockLoadCallback(gcbh);  FunctionName=sysgen  Parameters=ptable_  EnableBusSupport=off  mask(Xilinx Down Sampler Block){infoedit=Hardware notes: Sample and Latency controls determine the hardware implementation.  The cost in hardware of different implementations varies considerably; press Help for details., sample_ratio=2, sample_phase_sgadvanced=, sample_phase=Last Value of Frame  (most efficient), en_sgadvanced=, en=off, latency=1, dbl_ovrd_sgadvanced=, dbl_ovrd=off, xl_use_area_sgadvanced=, xl_use_area=off, xl_area=[0,0,0,0,0,0,0], has_advanced_control=0, sggui_pos=-1,-1,-1,-1, block_type=dsamp, block_version=, sg_icon_stat=60,56,1,1,white,blue,0,80c3f0cd,right,,[ ],[ ], sg_mask_display=|, sg_list_contents=, sg_blockgui_xml=}
      mask sg_mask_display=|
      | fprintf('','COMMENT: begin icon graphics');
      | patch([0 60 60 0 0 ],[0 0 56 56 0 ],[0.77 0.82 0.91 ]);
      | plot([0 60 60 0 0 ],[0 0 56 56 0 ]);
      | patch([12.2 23.76 31.76 39.76 47.76 31.76 20.2 12.2 ],[36.88 36.88 44.88 36.88 44.88 44.88 44.88 36.88 ],[1 1 1 ]);
      | patch([20.2 31.76 23.76 12.2 20.2 ],[28.88 28.88 36.88 36.88 28.88 ],[0.931 0.946 0.973 ]);
      | patch([12.2 23.76 31.76 20.2 12.2 ],[20.88 20.88 28.88 28.88 20.88 ],[1 1 1 ]);
      | patch([20.2 47.76 39.76 31.76 23.76 12.2 20.2 ],[12.88 12.88 20.88 12.88 20.88 20.88 12.88 ],[0.931 0.946 0.973 ]);
      | fprintf('','COMMENT: end icon graphics');
      | fprintf('','COMMENT: begin icon text');
      |
      |
      | color('black');disp('z^{-1}\newline ','texmode','on');
      | color('black');disp(' \newline{\fontsize{14pt}\bf\downarrow}2','texmode','on');
      | fprintf('','COMMENT: end icon text');
      mask prompts: infoedit ""; sample_ratio "Sampling rate (number of input samples per output sample)"; sample_phase_sgadvanced ""; sample_phase "Sample"; en_sgadvanced ""; en "Provide enable port"; dbl_ovrd_sgadvanced ""; dbl_ovrd "Override with doubles"; xl_use_area_sgadvanced ""; xl_use_area "Define FPGA area for resource estimation"; xl_area "FPGA area [slices, FFs, BRAMs, LUTs, IOBs, emb. mults, TBUFs]"; has_advanced_control ""; sggui_pos ""; block_type ""; block_version ""; sg_icon_stat ""; sg_mask_display ""; sg_list_contents ""; sg_blockgui_xml ""
      mask help: Hardware notes: Sample and Latency controls determine the hardware implementation. The cost in hardware of different implementations varies considerably; press Help for details.
      mask init:
      | try
      |   tmp_gcb = gcb;
      |   tmp_gcbh = gcbh;
      |   if (strcmp('SysGenIndex',get_param(bdroot(tmp_gcbh),'tag')) && ~isempty(regexp(bdroot(tmp_gcb), '^xbs', 'once')))
      |     return;
      |   end;
      |   xlMungeMaskParams;
      |   block_config = 'sysgen_blockset:Downsample_config';
      | 
      |   block_type='dsamp';
      | 
      |   serialized_declarations = '{''en''=>''Int'',''latency''=>''Int'',''sample_phase''=>''Int'',''sample_ratio''=>''Int'',''sim_engine''=>''Int'',''sysgen_root''=>''String'',''block_type''=>''String''}';
      |   xldsamp_init();
      |   ptable_ = xlblockprep(get_param(tmp_gcb, 'MaskWSVariables'));
      |   try
      |     xlBlockMoveCallback(tmp_gcbh);
      |   catch 
      |      clear global xl_updateicon_recursion_guard;
      |   end;
      | catch
      |   global dbgsysgen;
      |   if(~isempty(dbgsysgen) && dbgsysgen)
      |     e = regexprep(lasterr, '\n', '\nError: ');
      |     disp(['Error: While running MaskInit code on block ' tmp_gcb ': ' e]);
      |     error(e);
      |   end
      | end
      settings: CopyFcn=xlBlockMoveCallback(gcbh);  DeleteFcn=xlDestroyGui(gcbh);  ModelCloseFcn=xlDestroyGui(gcbh);  PreSaveFcn=xlBlockPreSaveCallback(gcbh);  PostSaveFcn=xlBlockPostSaveCallback(gcbh);  DestroyFcn=xlDestroyGui(gcbh);  OpenFcn=xlOpenGui(gcbh, 'dsamp_gui.xml', @xlmagicenablement, -1)  CloseFcn=xlDestroyGui(gcbh);  MoveFcn=xlBlockMoveCallback(gcbh);
      mask Help: eval('');xlDoc('-book','sysgen','-topic','Down_Sample');
      mask StyleString: edit,edit,edit,popup(First Value of Frame|Last Value of Frame  (most efficient)),edit,checkbox,edit,edit,checkbox,edit,checkbox,edit,edit,edit,edit,edit,edit,edit,edit,edit
      mask Display:
      | fprintf('','COMMENT: begin icon graphics');
      | patch([0 60 60 0 0 ],[0 0 56 56 0 ],[0.77 0.82 0.91 ]);
      | plot([0 60 60 0 0 ],[0 0 56 56 0 ]);
      | patch([12.2 23.76 31.76 39.76 47.76 31.76 20.2 12.2 ],[36.88 36.88 44.88 36.88 44.88 44.88 44.88 36.88 ],[1 1 1 ]);
      | patch([20.2 31.76 23.76 12.2 20.2 ],[28.88 28.88 36.88 36.88 28.88 ],[0.931 0.946 0.973 ]);
      | patch([12.2 23.76 31.76 20.2 12.2 ],[20.88 20.88 28.88 28.88 20.88 ],[1 1 1 ]);
      | patch([20.2 47.76 39.76 31.76 23.76 12.2 20.2 ],[12.88 12.88 20.88 12.88 20.88 20.88 12.88 ],[0.931 0.946 0.973 ]);
      | fprintf('','COMMENT: end icon graphics');
      | fprintf('','COMMENT: begin icon text');
      | 
      | 
      | color('black');disp('z^{-1}\newline ','texmode','on');
      | color('black');disp(' \newline{\fontsize{14pt}\bf\downarrow}2','texmode','on');
      | fprintf('','COMMENT: end icon text');
  Dual Port RAM : S-Function  LoadFcn=xlBlockLoadCallback(gcbh);  FunctionName=sysgen  Parameters=ptable_  EnableBusSupport=off  mask(Xilinx Dual Port Random Access Memory Block){depth=16, initVector=sin(pi*(0:15)/16), distributed_mem_sgadvanced=, distributed_mem=Block RAM, init_a=0, init_b=0, rst_a_sgadvanced=, rst_a=off, rst_b_sgadvanced=, rst_b=off, en_a_sgadvanced=, en_a=off, en_b_sgadvanced=, en_b=off, latency=1, write_mode_A_sgadvanced=, write_mode_A=Read After Write, write_mode_B_sgadvanced=, write_mode_B=Read After Write, dbl_ovrd_sgadvanced=, dbl_ovrd=off, optimize_sgadvanced=, optimize=Area, use_rpm_sgadvanced=, use_rpm=on, xl_use_area_sgadvanced=, xl_use_area=off, xl_area=[0,0,0,0,0,0,0], explicit_period=, period=, infoedit=, has_advanced_control=0, sggui_pos=-1,-1,-1,-1, block_type=dpram, block_version=, sg_icon_stat=75,165,6,2,white,blue,0,28af736d,right,,[ ],[ ], sg_mask_display=|, sg_list_contents=, sg_blockgui_xml=}
      mask sg_mask_display=|
      | fprintf('','COMMENT: begin icon graphics');
      | patch([0 75 75 0 0 ],[0 0 165 165 0 ],[0.77 0.82 0.91 ]);
      | plot([0 75 75 0 0 ],[0 0 165 165 0 ]);
      | patch([14.75 29.2 39.2 49.2 59.2 39.2 24.75 14.75 ],[93.1 93.1 103.1 93.1 103.1 103.1 103.1 93.1 ],[1 1 1 ]);
      | patch([24.75 39.2 29.2 14.75 24.75 ],[83.1 83.1 93.1 93.1 83.1 ],[0.931 0.946 0.973 ]);
      | patch([14.75 29.2 39.2 24.75 14.75 ],[73.1 73.1 83.1 83.1 73.1 ],[1 1 1 ]);
      | patch([24.75 59.2 49.2 39.2 29.2 14.75 24.75 ],[63.1 63.1 73.1 63.1 73.1 73.1 63.1 ],[0.931 0.946 0.973 ]);
      | fprintf('','COMMENT: end icon graphics');
      | fprintf('','COMMENT: begin icon text');
      | color('black');port_label('input',1,'addra');
      | color('black');port_label('input',2,'dina');
      | color('black');port_label('input',3,'wea');
      | color('black');port_label('input',4,'addrb');
      | color('black');port_label('input',5,'dinb');
      | color('black');port_label('input',6,'web');
      | color('black');port_label('output',1,'A');
      | color('black');port_label('output',2,'B');
      | fprintf('','COMMENT: end icon text');
      mask prompts: initVector "Initial value vector"; distributed_mem_sgadvanced ""; distributed_mem "Memory Type"; init_a "Initial value for port <tt>A</tt> output register"; init_b "Initial value for port <tt>B</tt> output register"; rst_a_sgadvanced ""; rst_a "Provide synchronous reset port for port <tt>A</tt> output register"; rst_b_sgadvanced ""; rst_b "Provide synchronous reset port for port <tt>B</tt> output register"; en_a_sgadvanced ""; en_a "Provide enable port for port <tt>A</tt>"; en_b_sgadvanced ""; en_b "Provide enable port for port <tt>B</tt>"; write_mode_A_sgadvanced ""; write_mode_A "Port <tt>A</tt>"; write_mode_B_sgadvanced ""; write_mode_B "Port <tt>B</tt>"; dbl_ovrd_sgadvanced ""; dbl_ovrd "Override with doubles"; optimize_sgadvanced ""; optimize "Optimize for"; use_rpm_sgadvanced ""; use_rpm "Use core placement information"; xl_use_area_sgadvanced ""; xl_use_area "Define FPGA area for resource estimation"; xl_area "FPGA area [slices, FFs, BRAMs, LUTs, IOBs, emb. mults, TBUFs]"; explicit_period ""; period ""; infoedit ""; has_advanced_control ""; sggui_pos ""; block_type ""; block_version ""; sg_icon_stat ""; sg_mask_display ""; sg_list_contents ""; sg_blockgui_xml ""
      mask help: Xilinx Dual Port Random Access Memory
      mask init:
      | try
      |   tmp_gcb = gcb;
      |   tmp_gcbh = gcbh;
      |   if (strcmp('SysGenIndex',get_param(bdroot(tmp_gcbh),'tag')) && ~isempty(regexp(bdroot(tmp_gcb), '^xbs', 'once')))
      |     return;
      |   end;
      |   xlMungeMaskParams;
      |   block_config = 'sysgen_blockset:Dpram_config';
      | 
      |   block_type='dpram';
      | 
      |   serialized_declarations = '{''dblOvrd''=>''Int'',''depth''=>''Int'',''distributed_mem''=>''Int'',''en_a''=>''Int'',''en_b''=>''Int'',''init''=>''DoubleVector'',''initVector''=>''DoubleVector'',''init_a''=>''Double'',''init_b''=>''Double'',''latency''=>''Int'',''optimize''=>''Int'',''rst_a''=>''Int'',''rst_b''=>''Int'',''sim_engine''=>''Int'',''use_rpm''=>''Int'',''write_mode_A''=>''Int'',''write_mode_B''=>''Int'',''write_mode_a''=>''Int'',''write_mode_b''=>''Int'',''block_type''=>''String''}';
      |   xldpram_init();
      |   ptable_ = xlblockprep(get_param(tmp_gcb, 'MaskWSVariables'));
      |   try
      |     xlBlockMoveCallback(tmp_gcbh);
      |   catch 
      |      clear global xl_updateicon_recursion_guard;
      |   end;
      | catch
      |   global dbgsysgen;
      |   if(~isempty(dbgsysgen) && dbgsysgen)
      |     e = regexprep(lasterr, '\n', '\nError: ');
      |     disp(['Error: While running MaskInit code on block ' tmp_gcb ': ' e]);
      |     error(e);
      |   end
      | end
      settings: CopyFcn=xlBlockMoveCallback(gcbh);  DeleteFcn=xlDestroyGui(gcbh);  ModelCloseFcn=xlDestroyGui(gcbh);  PreSaveFcn=xlBlockPreSaveCallback(gcbh);  PostSaveFcn=xlBlockPostSaveCallback(gcbh);  DestroyFcn=xlDestroyGui(gcbh);  OpenFcn=xlOpenGui(gcbh, 'dpram_gui.xml', @dpramenablement, -1)  CloseFcn=xlDestroyGui(gcbh);  MoveFcn=xlBlockMoveCallback(gcbh);
      mask Help: eval('');xlDoc('-book','sysgen','-topic','Dual_Port_RAM');
      mask StyleString: edit,edit,edit,popup(Distributed memory|Block RAM),edit,edit,edit,checkbox,edit,checkbox,edit,checkbox,edit,checkbox,edit,edit,popup(Read After Write|Read Before Write|No Read On Write),edit,popup(Read After Write|Read Before Write|No Read On Write),edit,checkbox,edit,popup(Area|Speed|Power),edit,checkbox,edit,checkbox,edit,edit,edit,edit,edit,edit,edit,edit,edit,edit,edit,edit
      mask Display:
      | fprintf('','COMMENT: begin icon graphics');
      | patch([0 75 75 0 0 ],[0 0 165 165 0 ],[0.77 0.82 0.91 ]);
      | plot([0 75 75 0 0 ],[0 0 165 165 0 ]);
      | patch([14.75 29.2 39.2 49.2 59.2 39.2 24.75 14.75 ],[93.1 93.1 103.1 93.1 103.1 103.1 103.1 93.1 ],[1 1 1 ]);
      | patch([24.75 39.2 29.2 14.75 24.75 ],[83.1 83.1 93.1 93.1 83.1 ],[0.931 0.946 0.973 ]);
      | patch([14.75 29.2 39.2 24.75 14.75 ],[73.1 73.1 83.1 83.1 73.1 ],[1 1 1 ]);
      | patch([24.75 59.2 49.2 39.2 29.2 14.75 24.75 ],[63.1 63.1 73.1 63.1 73.1 73.1 63.1 ],[0.931 0.946 0.973 ]);
      | fprintf('','COMMENT: end icon graphics');
      | fprintf('','COMMENT: begin icon text');
      | color('black');port_label('input',1,'addra');
      | color('black');port_label('input',2,'dina');
      | color('black');port_label('input',3,'wea');
      | color('black');port_label('input',4,'addrb');
      | color('black');port_label('input',5,'dinb');
      | color('black');port_label('input',6,'web');
      | color('black');port_label('output',1,'A');
      | color('black');port_label('output',2,'B');
      | fprintf('','COMMENT: end icon text');
  EDK Processor : Subsystem  LoadFcn=xlBlockLoadCallback(gcbh);  mask(Xilinx EDK Processor Block){mode=EDK pcore generation, xmp=, MemVisToProc=<qt bgcolor="#FFFFFF"></qt>, AvailableMemories=, portInterfaceTable=, bus_type_sgadvanced=, bus_type=AXI, baseaddr=0x80000000, baseaddr_lock_sgadvanced=, baseaddr_lock=off, dual_clock_sgadvanced=, dual_clock=on, reg_readback_sgadvanced=, reg_readback=off, ucf_file=, inheritDeviceType_sgadvanced=, inheritDeviceType=off, elf_file=, codebug_sgadvanced=, codebug=on, clock_name=plb, internalPortList={}, resetPolarity=0, memxtable={'mladdr'=>[],'mlist'=>[],'mlname'=>[],'mlstate'=>[]}, procinfo={}, memmapdirty=, blockname=, xpsintstyle=default, has_advanced_control=0, sggui_pos=-1,-1,-1,-1, block_type=edkprocessor, block_version=2.7, sg_icon_stat=62,64,-1,-1,white,blue,0,07734,right,,[ ],[ ], sg_mask_display=|, sg_list_contents={'table'=>{'AvailableMemories'=>'popup(<empty>)'}}, sg_blockgui_xml=}
      mask sg_mask_display=|
      | fprintf('','COMMENT: begin icon graphics');
      | patch([0 62 62 0 0 ],[0 0 64 64 0 ],[0.77 0.82 0.91 ]);
      | plot([0 62 62 0 0 ],[0 0 64 64 0 ]);
      | patch([13.2 24.76 32.76 40.76 48.76 32.76 21.2 13.2 ],[40.88 40.88 48.88 40.88 48.88 48.88 48.88 40.88 ],[1 1 1 ]);
      | patch([21.2 32.76 24.76 13.2 21.2 ],[32.88 32.88 40.88 40.88 32.88 ],[0.931 0.946 0.973 ]);
      | patch([13.2 24.76 32.76 21.2 13.2 ],[24.88 24.88 32.88 32.88 24.88 ],[1 1 1 ]);
      | patch([21.2 48.76 40.76 32.76 24.76 13.2 21.2 ],[16.88 16.88 24.88 16.88 24.88 24.88 16.88 ],[0.931 0.946 0.973 ]);
      | fprintf('','COMMENT: end icon graphics');
      | fprintf('','COMMENT: begin icon text');
      | fprintf('','COMMENT: end icon text');
      mask prompts: mode "Configure Processor for"; xmp "XPS Project"; MemVisToProc ""; AvailableMemories "Available Memories"; portInterfaceTable ""; bus_type_sgadvanced ""; bus_type "Bus Type"; baseaddr "Base Address"; baseaddr_lock_sgadvanced ""; baseaddr_lock "Lock"; dual_clock_sgadvanced ""; dual_clock "Dual Clocks"; reg_readback_sgadvanced ""; reg_readback "Register Read-Back"; ucf_file "Constraint File"; inheritDeviceType_sgadvanced ""; inheritDeviceType "Inherit Device Type"; elf_file "Initial Program"; codebug_sgadvanced ""; codebug "Enable Co-Debug with Xilinx SDK (Beta)"; clock_name ""; internalPortList ""; resetPolarity ""; memxtable ""; procinfo ""; memmapdirty ""; blockname ""; xpsintstyle ""; has_advanced_control ""; sggui_pos ""; block_type ""; block_version ""; sg_icon_stat ""; sg_mask_display ""; sg_list_contents ""; sg_blockgui_xml ""
      mask help: Xilinx EDK Processor
      mask init:
      | try
      |   tmp_gcb = gcb;
      |   tmp_gcbh = gcbh;
      |   if (strcmp('SysGenIndex',get_param(bdroot(tmp_gcbh),'tag')) && ~isempty(regexp(bdroot(tmp_gcb), '^xbs', 'once')))
      |     return;
      |   end;
      |   xlMungeMaskParams;
      | 
      |   block_type='edkprocessor';
      | 
      |   serialized_declarations = '{''block_type''=>''String''}';
      |   xledkprocessor_init();
      |   ptable_ = xlblockprep(get_param(tmp_gcb, 'MaskWSVariables'));
      |   try
      |     xlBlockMoveCallback(tmp_gcbh);
      |   catch 
      |      clear global xl_updateicon_recursion_guard;
      |   end;
      | catch
      |   global dbgsysgen;
      |   if(~isempty(dbgsysgen) && dbgsysgen)
      |     e = regexprep(lasterr, '\n', '\nError: ');
      |     disp(['Error: While running MaskInit code on block ' tmp_gcb ': ' e]);
      |     error(e);
      |   end
      | end
      settings: CopyFcn=xlProcBlockCopyCallback(gcbh);xlBlockMoveCallback(gcbh);  DeleteFcn=xlDestroyGui(gcbh);  ModelCloseFcn=xlDestroyGui(gcbh);  PreSaveFcn=xlBlockPreSaveCallback(gcbh);  PostSaveFcn=xlBlockPostSaveCallback(gcbh);  DestroyFcn=xlDestroyGui(gcbh);  OpenFcn=bh=gcbh;xlProcBlockCallbacks('populatesharedmemorylistbox',bh);xlOpenGui(bh, 'edkprocessor_gui.xml', @xlProcBlockEnablement, @xlProcBlockAction);  CloseFcn=xlDestroyGui(gcbh);  MoveFcn=xlBlockMoveCallback(gcbh);
      mask Help: eval('');xlDoc('-book','sysgen','-topic','EDK_Processor');
      mask StyleString: popup(EDK pcore generation|HDL netlisting),edit,edit,edit,edit,edit,popup(AXI|PLB),edit,edit,checkbox,edit,checkbox,edit,checkbox,edit,edit,checkbox,edit,edit,checkbox,edit,edit,edit,edit,edit,edit,edit,edit,edit,edit,edit,edit,edit,edit,edit,edit
      mask Display:
      | fprintf('','COMMENT: begin icon graphics');
      | patch([0 62 62 0 0 ],[0 0 64 64 0 ],[0.77 0.82 0.91 ]);
      | plot([0 62 62 0 0 ],[0 0 64 64 0 ]);
      | patch([13.2 24.76 32.76 40.76 48.76 32.76 21.2 13.2 ],[40.88 40.88 48.88 40.88 48.88 48.88 48.88 40.88 ],[1 1 1 ]);
      | patch([21.2 32.76 24.76 13.2 21.2 ],[32.88 32.88 40.88 40.88 32.88 ],[0.931 0.946 0.973 ]);
      | patch([13.2 24.76 32.76 21.2 13.2 ],[24.88 24.88 32.88 32.88 24.88 ],[1 1 1 ]);
      | patch([21.2 48.76 40.76 32.76 24.76 13.2 21.2 ],[16.88 16.88 24.88 16.88 24.88 24.88 16.88 ],[0.931 0.946 0.973 ]);
      | fprintf('','COMMENT: end icon graphics');
      | fprintf('','COMMENT: begin icon text');
      | fprintf('','COMMENT: end icon text');
